simulink model "hcu_main_ADASwEPS"  (Simulink 8.2)
settings: Solver=FixedStepDiscrete  StartTime=0.0  StopTime=inf  FixedStep=0.001  RelTol=1e-3
PostLoadFcn:
  | , if any(exist('dsrtsu_mdlpostloadfcn', 'file') == [2, 3, 6]), try dsrtsu_mdlpostloadfcn('Execute', bdroot); catch fprintf('Error in PostLoadFcn (dsrtsu_mdlpostloadfcn) for model "%s":\n %s\n', bdroot, lasterr); end, end,
values from neighbouring files (symbols this model uses):
  C_TASK_1MS_S = (	C_TICK_TIME_S       )    [hcu_local_hdr.m]    (also in temp_ovrd_values.m = double(	0.001                  ))
  C_TICK_TIME_S = single(	0.005	    	)    [hcu_local_hdr.m]
  ENUM_EPSLFCSTATUS_ACTIVE = uint8(  2  )    [hcu_local_hdr.m]
  ENUM_EPSLFCSTATUS_TRANSITION = uint8(  3  )    [hcu_local_hdr.m]
  ENUM_EPSLKASTATUS_ACTIVE = uint8(  2  )    [hcu_local_hdr.m]
  ENUM_EPSMODEREQ_ANGLE = uint8(  1  )    [hcu_local_hdr.m]
  ENUM_EPSMODEREQ_INTERNAL = uint8(  0  )    [hcu_local_hdr.m]
  ENUM_EPSMODEREQ_TORQUE = uint8(  2  )    [hcu_local_hdr.m]
  ENUM_GEARPOSN_1ST = uint8(  1  )    [hcu_local_hdr.m]
  ENUM_GEARPOSN_2ND = uint8(  2  )    [hcu_local_hdr.m]
  ENUM_GEARPOSN_3RD = uint8(  3  )    [hcu_local_hdr.m]
  ENUM_GEARPOSN_4TH = uint8(  4  )    [hcu_local_hdr.m]
  ENUM_GEARPOSN_5TH = uint8(  5  )    [hcu_local_hdr.m]
  ENUM_GEARPOSN_6TH = uint8(  6  )    [hcu_local_hdr.m]
  ENUM_GEARPOSN_R = uint8(  7  )    [hcu_local_hdr.m]
  FALSE = boolean( 0 )    [hcu_local_hdr.m]
  TRUE = boolean( 1 )    [hcu_local_hdr.m]
undefined symbols (not defined in the file or in its folder): AISP_EPSCurrent_pct, AISP_TqASensorDelta_pct, AISP_TqBSensorDelta_pct, dHAL_IN, hal, INVALID_ABS1_TIMEOUT, INVALID_ABS2_TIMEOUT, INVALID_ABS3_TIMEOUT, INVALID_ABS4_TIMEOUT, INVALID_AC1_TIMEOUT, INVALID_ADASTORQ_REQ, INVALID_BCM1_TIMEOUT, INVALID_BCM2_TIMEOUT, INVALID_BOOSTER_VAC, INVALID_CSW1_TIMEOUT, INVALID_CUR_VEHDECE, INVALID_CURBRAKEDECE_REQ, INVALID_CURSTEERANG_REQ, INVALID_CURSTEERTQ_REQ, INVALID_ECM1_TIMEOUT, INVALID_ECM2_TIMEOUT, INVALID_ECM3_TIMEOUT, INVALID_ECM9_TIMEOUT, INVALID_ENG_TORQUE_FRICTIONAL, INVALID_ENG_TORQUE_INDICATED, INVALID_ENG_TORQUE_INDICATEDCOR, INVALID_ENG_TQ_MAX, INVALID_ENG_TQ_MIN, INVALID_EPAS2_TIMEOUT, INVALID_EPAS3_TIMEOUT, INVALID_EPB1_TIMEOUT, INVALID_EPS_BATTVOLT, INVALID_ESC_BATTVOLT, INVALID_GRADE, INVALID_HCU3_TIMEOUT, INVALID_HCU4_TIMEOUT, INVALID_HMI1_TIMEOUT, INVALID_HMI2_TIMEOUT, INVALID_LAT_ACC, INVALID_LONG_ACC, INVALID_MC_PRESSURE, INVALID_METER1_TIMEOUT, INVALID_METER3_TIMEOUT, INVALID_METER_VEHSPD, INVALID_ODO_METER, INVALID_OUTSIDE_TEMP, INVALID_PARKBRAKEBIND_STAT, INVALID_PEDALTQ_REQ, INVALID_SAS1_TIMEOUT, INVALID_SAS_ANGLE, INVALID_SHIFTER_POSN, INVALID_TCM1_TIMEOUT, INVALID_TCM2_TIMEOUT, INVALID_VCU1_TIMEOUT, INVALID_VCU2_TIMEOUT, INVALID_VEH_CRASH, INVALID_VEH_SPD, INVALID_WHEEL_SPD, INVALID_YAW_RATE, KHAL_MssgIdObj1_num ... (+8)
libraries: simulink x147, hcu_lib x38, rti1401lib_dio_type3 x4, rtimmsu_dsrtlib x3, app x1, rtiethernetudplib x1, rti1401lib_adc_type4 x1, rti1401lib_dac_type3 x1, inp x1, lidr x1, outp x1
(part 5 of 15)

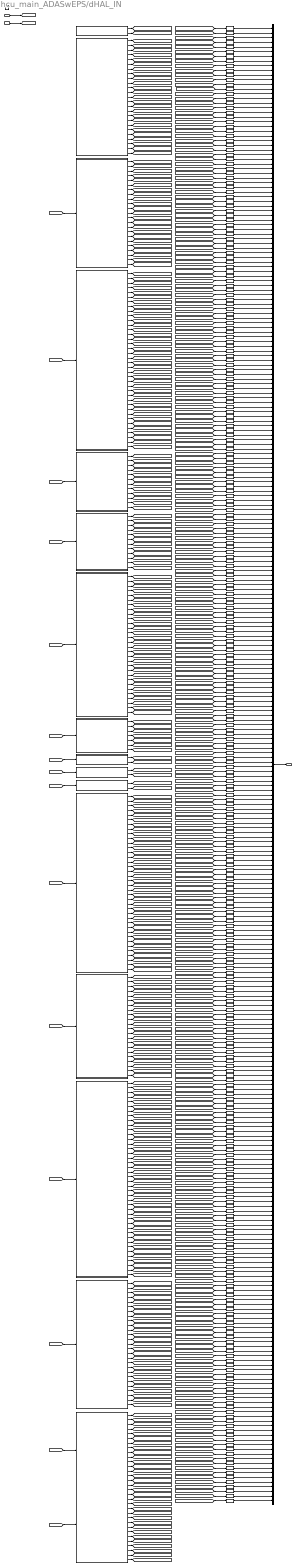
== system hcu_main_ADASwEPS/dHAL_IN ==
  CAN1_Rx : Inport
  CAN2_Rx : Inport  Port=2
  trig_dhal_in : TriggerPort  TriggerType=function-call
  ABS1RollCntCvt : DataTypeConversion  OutDataTypeStr=uint8  SaturateOnIntegerOverflow=on  RndMeth=Zero
  ABS2ChkSumValidCvt : DataTypeConversion  OutDataTypeStr=boolean  SaturateOnIntegerOverflow=on  RndMeth=Zero
  ABS2RollCntCvt : DataTypeConversion  OutDataTypeStr=uint8  SaturateOnIntegerOverflow=on  RndMeth=Zero
  ABSActiveCvt : DataTypeConversion  OutDataTypeStr=boolean  SaturateOnIntegerOverflow=on  RndMeth=Zero
  ABSFaultCvt : DataTypeConversion  OutDataTypeStr=boolean  SaturateOnIntegerOverflow=on  RndMeth=Zero
  ACCCancelHCvt : DataTypeConversion  OutDataTypeStr=boolean  SaturateOnIntegerOverflow=on  RndMeth=Zero
  ACCOnHCvt : DataTypeConversion  OutDataTypeStr=boolean  SaturateOnIntegerOverflow=on  RndMeth=Zero
  ACCOnVCUCvt : DataTypeConversion  OutDataTypeStr=boolean  SaturateOnIntegerOverflow=on  RndMeth=Zero
  ACCResSpdIncHCvt : DataTypeConversion  OutDataTypeStr=boolean  SaturateOnIntegerOverflow=on  RndMeth=Zero
  ACCResSpdIncVCUCvt : DataTypeConversion  OutDataTypeStr=boolean  SaturateOnIntegerOverflow=on  RndMeth=Zero
  ACCSetSpdDecHCvt : DataTypeConversion  OutDataTypeStr=boolean  SaturateOnIntegerOverflow=on  RndMeth=Zero
  ACCSetSpdDecVCUCvt : DataTypeConversion  OutDataTypeStr=boolean  SaturateOnIntegerOverflow=on  RndMeth=Zero
  ACCSpdDecHCvt : DataTypeConversion  OutDataTypeStr=boolean  SaturateOnIntegerOverflow=on  RndMeth=Zero
  ACCSpdIncHCvt : DataTypeConversion  OutDataTypeStr=boolean  SaturateOnIntegerOverflow=on  RndMeth=Zero
  ACCTimeGapDecHCvt : DataTypeConversion  OutDataTypeStr=boolean  SaturateOnIntegerOverflow=on  RndMeth=Zero
  ACCTimeGapDecVCUCvt : DataTypeConversion  OutDataTypeStr=boolean  SaturateOnIntegerOverflow=on  RndMeth=Zero
  ACCTimeGapIncHCvt : DataTypeConversion  OutDataTypeStr=boolean  SaturateOnIntegerOverflow=on  RndMeth=Zero
  ACCTimeGapIncVCUCvt : DataTypeConversion  OutDataTypeStr=boolean  SaturateOnIntegerOverflow=on  RndMeth=Zero
  ADCFaultCvt : DataTypeConversion  OutDataTypeStr=uint8  SaturateOnIntegerOverflow=on  RndMeth=Zero
  AEBEnableHCvt : DataTypeConversion  OutDataTypeStr=boolean  SaturateOnIntegerOverflow=on  RndMeth=Zero
  AccelPedalPosnCvt : DataTypeConversion  OutDataTypeStr=single  SaturateOnIntegerOverflow=on  RndMeth=Zero
  AccelPedalPosnInvalidCvt : DataTypeConversion  OutDataTypeStr=boolean  SaturateOnIntegerOverflow=on  RndMeth=Zero
  AckCurBrakDecReqApplableCvt : DataTypeConversion  OutDataTypeStr=boolean  SaturateOnIntegerOverflow=on  RndMeth=Zero
  AckCurBrakDecReqCvt : DataTypeConversion  OutDataTypeStr=single  SaturateOnIntegerOverflow=on  RndMeth=Zero
  AckCurBrakDecReqInvalidCvt : DataTypeConversion  OutDataTypeStr=boolean  SaturateOnIntegerOverflow=on  RndMeth=Zero
  AckCurPTTqReqApplableCvt : DataTypeConversion  OutDataTypeStr=boolean  SaturateOnIntegerOverflow=on  RndMeth=Zero
  AckCurPTTqReqCvt : DataTypeConversion  OutDataTypeStr=single  SaturateOnIntegerOverflow=on  RndMeth=Zero
  AckCurPTTqReqInvalidCvt : DataTypeConversion  OutDataTypeStr=boolean  SaturateOnIntegerOverflow=on  RndMeth=Zero
  AckCurStrAngReqApplableCvt : DataTypeConversion  OutDataTypeStr=boolean  SaturateOnIntegerOverflow=on  RndMeth=Zero
  AckCurStrAngReqCvt : DataTypeConversion  OutDataTypeStr=single  SaturateOnIntegerOverflow=on  RndMeth=Zero
  AckCurStrAngReqInvalidCvt : DataTypeConversion  OutDataTypeStr=boolean  SaturateOnIntegerOverflow=on  RndMeth=Zero
  AckCurStrTqReqApplableCvt : DataTypeConversion  OutDataTypeStr=boolean  SaturateOnIntegerOverflow=on  RndMeth=Zero
  AckCurStrTqReqCvt : DataTypeConversion  OutDataTypeStr=single  SaturateOnIntegerOverflow=on  RndMeth=Zero
  AckCurStrTqReqInvalidCvt : DataTypeConversion  OutDataTypeStr=boolean  SaturateOnIntegerOverflow=on  RndMeth=Zero
  AckCurVehDecCvt : DataTypeConversion  OutDataTypeStr=single  SaturateOnIntegerOverflow=on  RndMeth=Zero
  AckCurVehDecInvalidCvt : DataTypeConversion  OutDataTypeStr=boolean  SaturateOnIntegerOverflow=on  RndMeth=Zero
  AnyDoorOpenCvt : DataTypeConversion  OutDataTypeStr=boolean  SaturateOnIntegerOverflow=on  RndMeth=Zero
  AppTimeCvt : DataTypeConversion  OutDataTypeStr=single  SaturateOnIntegerOverflow=on  RndMeth=Zero
  BrakBoosterPresCvt : DataTypeConversion  OutDataTypeStr=single  SaturateOnIntegerOverflow=on  RndMeth=Zero
  BrakBoosterPresInvalidCvt : DataTypeConversion  OutDataTypeStr=boolean  SaturateOnIntegerOverflow=on  RndMeth=Zero
  BrkLampOnCvt : DataTypeConversion  OutDataTypeStr=boolean  SaturateOnIntegerOverflow=on  RndMeth=Zero
  BrkLampSigInvalidCvt : DataTypeConversion  OutDataTypeStr=boolean  SaturateOnIntegerOverflow=on  RndMeth=Zero
  BuzzerSwOnFltOpenCircuitCvt : DataTypeConversion  OutDataTypeStr=uint8  SaturateOnIntegerOverflow=on  RndMeth=Zero
  BuzzerSwOnFltShortHighCvt : DataTypeConversion  OutDataTypeStr=uint8  SaturateOnIntegerOverflow=on  RndMeth=Zero
  BuzzerSwOnFltShortLowCvt : DataTypeConversion  OutDataTypeStr=uint8  SaturateOnIntegerOverflow=on  RndMeth=Zero
  CANMsgValidABS1Cvt : DataTypeConversion  OutDataTypeStr=boolean  SaturateOnIntegerOverflow=on  RndMeth=Zero
  CANMsgValidABS2Cvt : DataTypeConversion  OutDataTypeStr=boolean  SaturateOnIntegerOverflow=on  RndMeth=Zero
  CANMsgValidABS3Cvt : DataTypeConversion  OutDataTypeStr=boolean  SaturateOnIntegerOverflow=on  RndMeth=Zero
  CANMsgValidABS4Cvt : DataTypeConversion  OutDataTypeStr=boolean  SaturateOnIntegerOverflow=on  RndMeth=Zero
  CANMsgValidAC1Cvt : DataTypeConversion  OutDataTypeStr=boolean  SaturateOnIntegerOverflow=on  RndMeth=Zero
  CANMsgValidBCM1Cvt : DataTypeConversion  OutDataTypeStr=boolean  SaturateOnIntegerOverflow=on  RndMeth=Zero
  CANMsgValidBCM2Cvt : DataTypeConversion  OutDataTypeStr=boolean  SaturateOnIntegerOverflow=on  RndMeth=Zero
  CANMsgValidECM1Cvt : DataTypeConversion  OutDataTypeStr=boolean  SaturateOnIntegerOverflow=on  RndMeth=Zero
  CANMsgValidECM2Cvt : DataTypeConversion  OutDataTypeStr=boolean  SaturateOnIntegerOverflow=on  RndMeth=Zero
  CANMsgValidECM3Cvt : DataTypeConversion  OutDataTypeStr=boolean  SaturateOnIntegerOverflow=on  RndMeth=Zero
  CANMsgValidECM9Cvt : DataTypeConversion  OutDataTypeStr=boolean  SaturateOnIntegerOverflow=on  RndMeth=Zero
  CANMsgValidEPAS1Cvt : DataTypeConversion  OutDataTypeStr=boolean  SaturateOnIntegerOverflow=on  RndMeth=Zero
  CANMsgValidEPAS2Cvt : DataTypeConversion  OutDataTypeStr=boolean  SaturateOnIntegerOverflow=on  RndMeth=Zero
  CANMsgValidEPAS3Cvt : DataTypeConversion  OutDataTypeStr=boolean  SaturateOnIntegerOverflow=on  RndMeth=Zero
  CANMsgValidEPB1Cvt : DataTypeConversion  OutDataTypeStr=boolean  SaturateOnIntegerOverflow=on  RndMeth=Zero
  CANMsgValidEPB1Cvt1 : DataTypeConversion  OutDataTypeStr=boolean  SaturateOnIntegerOverflow=on  RndMeth=Zero
  CANMsgValidEPM1Cvt : DataTypeConversion  OutDataTypeStr=boolean  SaturateOnIntegerOverflow=on  RndMeth=Zero
  CANMsgValidEPM2Cvt : DataTypeConversion  OutDataTypeStr=boolean  SaturateOnIntegerOverflow=on  RndMeth=Zero
  CANMsgValidEPM3Cvt : DataTypeConversion  OutDataTypeStr=boolean  SaturateOnIntegerOverflow=on  RndMeth=Zero
  CANMsgValidEPM4Cvt : DataTypeConversion  OutDataTypeStr=boolean  SaturateOnIntegerOverflow=on  RndMeth=Zero
  CANMsgValidEPM4Cvt1 : DataTypeConversion  OutDataTypeStr=boolean  SaturateOnIntegerOverflow=on  RndMeth=Zero
  CANMsgValidHCU3Cvt : DataTypeConversion  OutDataTypeStr=boolean  SaturateOnIntegerOverflow=on  RndMeth=Zero
  CANMsgValidHCU4Cvt : DataTypeConversion  OutDataTypeStr=boolean  SaturateOnIntegerOverflow=on  RndMeth=Zero
  CANMsgValidHMI1Cvt : DataTypeConversion  OutDataTypeStr=boolean  SaturateOnIntegerOverflow=on  RndMeth=Zero
  CANMsgValidHMI2Cvt : DataTypeConversion  OutDataTypeStr=boolean  SaturateOnIntegerOverflow=on  RndMeth=Zero
  CANMsgValidMETER1Cvt : DataTypeConversion  OutDataTypeStr=boolean  SaturateOnIntegerOverflow=on  RndMeth=Zero
  CANMsgValidMETER3Cvt : DataTypeConversion  OutDataTypeStr=boolean  SaturateOnIntegerOverflow=on  RndMeth=Zero
  CANMsgValidSAS1Cvt : DataTypeConversion  OutDataTypeStr=boolean  SaturateOnIntegerOverflow=on  RndMeth=Zero
  CANMsgValidTCM1Cvt : DataTypeConversion  OutDataTypeStr=boolean  SaturateOnIntegerOverflow=on  RndMeth=Zero
  CANMsgValidTCM2Cvt : DataTypeConversion  OutDataTypeStr=boolean  SaturateOnIntegerOverflow=on  RndMeth=Zero
  CANMsgValidVCU1Cvt : DataTypeConversion  OutDataTypeStr=boolean  SaturateOnIntegerOverflow=on  RndMeth=Zero
  CANMsgValidVCU2Cvt : DataTypeConversion  OutDataTypeStr=boolean  SaturateOnIntegerOverflow=on  RndMeth=Zero
  CSCEnableHCvt : DataTypeConversion  OutDataTypeStr=boolean  SaturateOnIntegerOverflow=on  RndMeth=Zero
  CurDriverTqReqCvt : DataTypeConversion  OutDataTypeStr=single  SaturateOnIntegerOverflow=on  RndMeth=Zero
  CurDriverTqReqInvalidCvt : DataTypeConversion  OutDataTypeStr=boolean  SaturateOnIntegerOverflow=on  RndMeth=Zero
  CurDriverTqReqInvalidCvt1 : DataTypeConversion  OutDataTypeStr=uint8  SaturateOnIntegerOverflow=on  RndMeth=Zero
  DeceContManagCvt : DataTypeConversion  OutDataTypeStr=boolean  SaturateOnIntegerOverflow=on  RndMeth=Zero
  DefMaxACCSetSpeedCvt : DataTypeConversion  OutDataTypeStr=single  SaturateOnIntegerOverflow=on  RndMeth=Zero
  DriverBrakPedalOnCvt : DataTypeConversion  OutDataTypeStr=boolean  SaturateOnIntegerOverflow=on  RndMeth=Zero
  DriverBrakPedalOnCvt1 : DataTypeConversion  OutDataTypeStr=boolean  SaturateOnIntegerOverflow=on  RndMeth=Zero
  DriverDoorOpenCvt : DataTypeConversion  OutDataTypeStr=boolean  SaturateOnIntegerOverflow=on  RndMeth=Zero
  DriverModeCvt : DataTypeConversion  OutDataTypeStr=uint8  SaturateOnIntegerOverflow=on  RndMeth=Zero
  EBDFaultCvt : DataTypeConversion  OutDataTypeStr=boolean  SaturateOnIntegerOverflow=on  RndMeth=Zero
  ECM9RollCntCvt : DataTypeConversion  OutDataTypeStr=uint8  SaturateOnIntegerOverflow=on  RndMeth=Zero
  ECMExtnTqAvailableCvt : DataTypeConversion  OutDataTypeStr=boolean  SaturateOnIntegerOverflow=on  RndMeth=Zero
  ECMPermMaxTqIndCvt : DataTypeConversion  OutDataTypeStr=boolean  SaturateOnIntegerOverflow=on  RndMeth=Zero
  ECMTqSourceCvt : DataTypeConversion  OutDataTypeStr=uint8  SaturateOnIntegerOverflow=on  RndMeth=Zero
  EEPROMFaultCvt : DataTypeConversion  OutDataTypeStr=uint8  SaturateOnIntegerOverflow=on  RndMeth=Zero
  EMSHybridOpStateCvt : DataTypeConversion  OutDataTypeStr=uint8  SaturateOnIntegerOverflow=on  RndMeth=Zero
  EMSOpStateCvt : DataTypeConversion  OutDataTypeStr=uint8  SaturateOnIntegerOverflow=on  RndMeth=Zero
  EPAS2ChkSumValidCvt : DataTypeConversion  OutDataTypeStr=boolean  SaturateOnIntegerOverflow=on  RndMeth=Zero
  EPAS2RollCntCvt : DataTypeConversion  OutDataTypeStr=uint8  SaturateOnIntegerOverflow=on  RndMeth=Zero
  EPAS3ChkSumValidCvt : DataTypeConversion  OutDataTypeStr=boolean  SaturateOnIntegerOverflow=on  RndMeth=Zero
  EPAS3RollCntCvt{,2..4} (4 alike) : DataTypeConversion  OutDataTypeStr=uint8  SaturateOnIntegerOverflow=on  RndMeth=Zero
  EPASMILReqCvt : DataTypeConversion  OutDataTypeStr=boolean  SaturateOnIntegerOverflow=on  RndMeth=Zero
  EPSBattVoltCvt : DataTypeConversion  OutDataTypeStr=single  SaturateOnIntegerOverflow=on  RndMeth=Zero
  EPSBattVoltInvalidCvt : DataTypeConversion  OutDataTypeStr=boolean  SaturateOnIntegerOverflow=on  RndMeth=Zero
  EPSElectPWRCvt : DataTypeConversion  OutDataTypeStr=single  SaturateOnIntegerOverflow=on  RndMeth=Zero
  EPSFailedCvt : DataTypeConversion  OutDataTypeStr=boolean  SaturateOnIntegerOverflow=on  RndMeth=Zero
  ESCActiveCvt : DataTypeConversion  OutDataTypeStr=boolean  SaturateOnIntegerOverflow=on  RndMeth=Zero
  ESCBattVoltCvt : DataTypeConversion  OutDataTypeStr=single  SaturateOnIntegerOverflow=on  RndMeth=Zero
  ESCBattVoltInvalidCvt : DataTypeConversion  OutDataTypeStr=boolean  SaturateOnIntegerOverflow=on  RndMeth=Zero
  ESCBrakeStatusCvt : DataTypeConversion  OutDataTypeStr=uint8  SaturateOnIntegerOverflow=on  RndMeth=Zero
  ESCExtnBrkAvailableCvt : DataTypeConversion  OutDataTypeStr=boolean  SaturateOnIntegerOverflow=on  RndMeth=Zero
  ESCFaultCvt : DataTypeConversion  OutDataTypeStr=boolean  SaturateOnIntegerOverflow=on  RndMeth=Zero
  EffAccelPedalPosnCvt : DataTypeConversion  OutDataTypeStr=single  SaturateOnIntegerOverflow=on  RndMeth=Zero
  EffAccelPedalPosnInvalidCvt : DataTypeConversion  OutDataTypeStr=boolean  SaturateOnIntegerOverflow=on  RndMeth=Zero
  EngHoodOpenCvt : DataTypeConversion  OutDataTypeStr=boolean  SaturateOnIntegerOverflow=on  RndMeth=Zero
  EngRunningCvt : DataTypeConversion  OutDataTypeStr=boolean  SaturateOnIntegerOverflow=on  RndMeth=Zero
  EngRunningCvt1 : DataTypeConversion  OutDataTypeStr=boolean  SaturateOnIntegerOverflow=on  RndMeth=Zero
  EngSpdCvt : DataTypeConversion  OutDataTypeStr=single  SaturateOnIntegerOverflow=on  RndMeth=Zero
  EngSpdInvalidCvt : DataTypeConversion  OutDataTypeStr=boolean  SaturateOnIntegerOverflow=on  RndMeth=Zero
  EngTqFrictionCvt : DataTypeConversion  OutDataTypeStr=single  SaturateOnIntegerOverflow=on  RndMeth=Zero
  EngTqFrictionInvalidCvt : DataTypeConversion  OutDataTypeStr=boolean  SaturateOnIntegerOverflow=on  RndMeth=Zero
  EngTqIndicatedCORCvt : DataTypeConversion  OutDataTypeStr=single  SaturateOnIntegerOverflow=on  RndMeth=Zero
  EngTqIndicatedCORInvalidCvt : DataTypeConversion  OutDataTypeStr=boolean  SaturateOnIntegerOverflow=on  RndMeth=Zero
  EngTqIndicatedCvt : DataTypeConversion  OutDataTypeStr=single  SaturateOnIntegerOverflow=on  RndMeth=Zero
  EngTqIndicatedInvalidCvt : DataTypeConversion  OutDataTypeStr=boolean  SaturateOnIntegerOverflow=on  RndMeth=Zero
  EngTqMaxCvt : DataTypeConversion  OutDataTypeStr=single  SaturateOnIntegerOverflow=on  RndMeth=Zero
  EngTqMaxInvalidCvt : DataTypeConversion  OutDataTypeStr=boolean  SaturateOnIntegerOverflow=on  RndMeth=Zero
  EngTqMinCvt : DataTypeConversion  OutDataTypeStr=single  SaturateOnIntegerOverflow=on  RndMeth=Zero
  EngTqMinInvalidCvt : DataTypeConversion  OutDataTypeStr=boolean  SaturateOnIntegerOverflow=on  RndMeth=Zero
  EngTqUnCORFaultCvt : DataTypeConversion  OutDataTypeStr=boolean  SaturateOnIntegerOverflow=on  RndMeth=Zero
  FCWEnableHCvt : DataTypeConversion  OutDataTypeStr=boolean  SaturateOnIntegerOverflow=on  RndMeth=Zero
  FCWWarningModeHCvt : DataTypeConversion  OutDataTypeStr=uint8  SaturateOnIntegerOverflow=on  RndMeth=Zero
  HAL_IN_CANVALID : Subsystem
  HAL_IN_CSW : Subsystem
  HAL_IN_EPB : Subsystem
  HAL_IN_EPM : Subsystem
  HAL_IN_HMI : Subsystem
  HAL_IN_RadObjDecoder : Subsystem
  HAL_IN_VCU : Subsystem
  HCU3RollCntCvt : DataTypeConversion  OutDataTypeStr=uint8  SaturateOnIntegerOverflow=on  RndMeth=Zero
  HSAActiveCvt : DataTypeConversion  OutDataTypeStr=boolean  SaturateOnIntegerOverflow=on  RndMeth=Zero
  HSAFaultCvt : DataTypeConversion  OutDataTypeStr=boolean  SaturateOnIntegerOverflow=on  RndMeth=Zero
  HWAccelPedalPosnCvt : DataTypeConversion  OutDataTypeStr=single  SaturateOnIntegerOverflow=on  RndMeth=Zero
  HWAccelPedalPosnInvalidCvt : DataTypeConversion  OutDataTypeStr=boolean  SaturateOnIntegerOverflow=on  RndMeth=Zero
  HazardLightSwCvt : DataTypeConversion  OutDataTypeStr=boolean  SaturateOnIntegerOverflow=on  RndMeth=Zero
  IGSAOnHCvt : DataTypeConversion  OutDataTypeStr=boolean  SaturateOnIntegerOverflow=on  RndMeth=Zero
  IGSAResSpdIncHCvt : DataTypeConversion  OutDataTypeStr=boolean  SaturateOnIntegerOverflow=on  RndMeth=Zero
  IGSASetSpdDecHCvt : DataTypeConversion  OutDataTypeStr=boolean  SaturateOnIntegerOverflow=on  RndMeth=Zero
  IGSASwitchModeHCvt : DataTypeConversion  OutDataTypeStr=boolean  SaturateOnIntegerOverflow=on  RndMeth=Zero
  IgnitionVoltCvt : DataTypeConversion  OutDataTypeStr=single  SaturateOnIntegerOverflow=on  RndMeth=Zero
  KeySwitchStatusCvt : DataTypeConversion  OutDataTypeStr=uint8  SaturateOnIntegerOverflow=on  RndMeth=Zero
  LCSEnableHCvt : DataTypeConversion  OutDataTypeStr=boolean  SaturateOnIntegerOverflow=on  RndMeth=Zero
  LFCOnVCUCvt : DataTypeConversion  OutDataTypeStr=boolean  SaturateOnIntegerOverflow=on  RndMeth=Zero
  LFCPilotCancelHCvt : DataTypeConversion  OutDataTypeStr=boolean  SaturateOnIntegerOverflow=on  RndMeth=Zero
  LFCPilotOnHCvt : DataTypeConversion  OutDataTypeStr=boolean  SaturateOnIntegerOverflow=on  RndMeth=Zero
  LFWheelSpeedCvt : DataTypeConversion  OutDataTypeStr=single  SaturateOnIntegerOverflow=on  RndMeth=Zero
  LFWheelSpeedInvalidCvt : DataTypeConversion  OutDataTypeStr=boolean  SaturateOnIntegerOverflow=on  RndMeth=Zero
  LKAEnableHCvt : DataTypeConversion  OutDataTypeStr=boolean  SaturateOnIntegerOverflow=on  RndMeth=Zero
  LRDoorOpenCvt : DataTypeConversion  OutDataTypeStr=boolean  SaturateOnIntegerOverflow=on  RndMeth=Zero
  LRWheelSpeedCvt : DataTypeConversion  OutDataTypeStr=single  SaturateOnIntegerOverflow=on  RndMeth=Zero
  LRWheelSpeedInvalidCvt : DataTypeConversion  OutDataTypeStr=boolean  SaturateOnIntegerOverflow=on  RndMeth=Zero
  LampBlueOnFltOpenCircuitCvt : DataTypeConversion  OutDataTypeStr=uint8  SaturateOnIntegerOverflow=on  RndMeth=Zero
  LampBlueOnFltShortHighCvt : DataTypeConversion  OutDataTypeStr=uint8  SaturateOnIntegerOverflow=on  RndMeth=Zero
  LampBlueOnFltShortLowCvt : DataTypeConversion  OutDataTypeStr=uint8  SaturateOnIntegerOverflow=on  RndMeth=Zero
  LampGreenOnFltOpenCircuitCvt : DataTypeConversion  OutDataTypeStr=uint8  SaturateOnIntegerOverflow=on  RndMeth=Zero
  LampGreenOnFltShortHighCvt : DataTypeConversion  OutDataTypeStr=uint8  SaturateOnIntegerOverflow=on  RndMeth=Zero
  LampGreenOnFltShortLowCvt : DataTypeConversion  OutDataTypeStr=uint8  SaturateOnIntegerOverflow=on  RndMeth=Zero
  LampRedOnFltOpenCircuitCvt : DataTypeConversion  OutDataTypeStr=uint8  SaturateOnIntegerOverflow=on  RndMeth=Zero
  LampRedOnFltShortHighCvt : DataTypeConversion  OutDataTypeStr=uint8  SaturateOnIntegerOverflow=on  RndMeth=Zero
  LampRedOnFltShortLowCvt : DataTypeConversion  OutDataTypeStr=uint8  SaturateOnIntegerOverflow=on  RndMeth=Zero
  LampYellowOnFltOpenCircuitCvt : DataTypeConversion  OutDataTypeStr=uint8  SaturateOnIntegerOverflow=on  RndMeth=Zero
  LampYellowOnFltShortHighCvt : DataTypeConversion  OutDataTypeStr=uint8  SaturateOnIntegerOverflow=on  RndMeth=Zero
  LampYellowOnFltShortLowCvt : DataTypeConversion  OutDataTypeStr=uint8  SaturateOnIntegerOverflow=on  RndMeth=Zero
  LaneC0LCvt : DataTypeConversion  OutDataTypeStr=single  SaturateOnIntegerOverflow=on  RndMeth=Zero
  LaneC0RCvt : DataTypeConversion  OutDataTypeStr=single  SaturateOnIntegerOverflow=on  RndMeth=Zero
  LaneC1LCvt : DataTypeConversion  OutDataTypeStr=single  SaturateOnIntegerOverflow=on  RndMeth=Zero
  LaneC1RCvt : DataTypeConversion  OutDataTypeStr=single  SaturateOnIntegerOverflow=on  RndMeth=Zero
  LaneC2LCvt : DataTypeConversion  OutDataTypeStr=single  SaturateOnIntegerOverflow=on  RndMeth=Zero
  LaneC2RCvt : DataTypeConversion  OutDataTypeStr=single  SaturateOnIntegerOverflow=on  RndMeth=Zero
  LaneC3LCvt : DataTypeConversion  OutDataTypeStr=single  SaturateOnIntegerOverflow=on  RndMeth=Zero
  LaneC3RCvt : DataTypeConversion  OutDataTypeStr=single  SaturateOnIntegerOverflow=on  RndMeth=Zero
  LaneCrosLCvt : DataTypeConversion  OutDataTypeStr=boolean  SaturateOnIntegerOverflow=on  RndMeth=Zero
  LaneCrosRCvt : DataTypeConversion  OutDataTypeStr=boolean  SaturateOnIntegerOverflow=on  RndMeth=Zero
  LaneMrkClrLCvt : DataTypeConversion  OutDataTypeStr=uint8  SaturateOnIntegerOverflow=on  RndMeth=Zero
  LaneMrkClrRCvt : DataTypeConversion  OutDataTypeStr=uint8  SaturateOnIntegerOverflow=on  RndMeth=Zero
  LaneMrkWidLCvt : DataTypeConversion  OutDataTypeStr=single  SaturateOnIntegerOverflow=on  RndMeth=Zero
  LaneMrkWidRCvt : DataTypeConversion  OutDataTypeStr=single  SaturateOnIntegerOverflow=on  RndMeth=Zero
  LaneQualityLCvt : DataTypeConversion  OutDataTypeStr=uint8  SaturateOnIntegerOverflow=on  RndMeth=Zero
  LaneQualityRCvt : DataTypeConversion  OutDataTypeStr=uint8  SaturateOnIntegerOverflow=on  RndMeth=Zero
  LaneTypeLCvt : DataTypeConversion  OutDataTypeStr=uint8  SaturateOnIntegerOverflow=on  RndMeth=Zero
  LaneTypeRCvt : DataTypeConversion  OutDataTypeStr=uint8  SaturateOnIntegerOverflow=on  RndMeth=Zero
  LatAccelCvt : DataTypeConversion  OutDataTypeStr=single  SaturateOnIntegerOverflow=on  RndMeth=Zero
  LatAccelInvalidCvt : DataTypeConversion  OutDataTypeStr=boolean  SaturateOnIntegerOverflow=on  RndMeth=Zero
  LatDistToborderLeftCvt : DataTypeConversion  OutDataTypeStr=single  SaturateOnIntegerOverflow=on  RndMeth=Zero
  LatDistToborderRightCvt : DataTypeConversion  OutDataTypeStr=single  SaturateOnIntegerOverflow=on  RndMeth=Zero
  LongAccelCvt : DataTypeConversion  OutDataTypeStr=single  SaturateOnIntegerOverflow=on  RndMeth=Zero
  LongAccelInvalidCvt : DataTypeConversion  OutDataTypeStr=boolean  SaturateOnIntegerOverflow=on  RndMeth=Zero
  LowBrakBoosterPresCvt : DataTypeConversion  OutDataTypeStr=boolean  SaturateOnIntegerOverflow=on  RndMeth=Zero
  LowBrakeFluidCvt : DataTypeConversion  OutDataTypeStr=boolean  SaturateOnIntegerOverflow=on  RndMeth=Zero
  MAPAEnableHCvt : DataTypeConversion  OutDataTypeStr=boolean  SaturateOnIntegerOverflow=on  RndMeth=Zero
  MCPressureCvt : DataTypeConversion  OutDataTypeStr=single  SaturateOnIntegerOverflow=on  RndMeth=Zero
  MCPressureInvalidCvt : DataTypeConversion  OutDataTypeStr=boolean  SaturateOnIntegerOverflow=on  RndMeth=Zero
  MILReqCvt : DataTypeConversion  OutDataTypeStr=boolean  SaturateOnIntegerOverflow=on  RndMeth=Zero
  MSAOnVCUCvt : DataTypeConversion  OutDataTypeStr=boolean  SaturateOnIntegerOverflow=on  RndMeth=Zero
  MeasCounterCvt : DataTypeConversion  OutDataTypeStr=uint8  SaturateOnIntegerOverflow=on  RndMeth=Zero
  MeterVehSpdCvt : DataTypeConversion  OutDataTypeStr=single  SaturateOnIntegerOverflow=on  RndMeth=Zero
  MeterVehSpdInvalidCvt : DataTypeConversion  OutDataTypeStr=boolean  SaturateOnIntegerOverflow=on  RndMeth=Zero
  NowGearPosnCvt : DataTypeConversion  OutDataTypeStr=uint8  SaturateOnIntegerOverflow=on  RndMeth=Zero
  NowGearPosnInvalidCvt : DataTypeConversion  OutDataTypeStr=boolean  SaturateOnIntegerOverflow=on  RndMeth=Zero
  OBUBuzzerOnFltOpenCircuitCvt : DataTypeConversion  OutDataTypeStr=uint8  SaturateOnIntegerOverflow=on  RndMeth=Zero
  OBUBuzzerOnFltShortHighCvt : DataTypeConversion  OutDataTypeStr=uint8  SaturateOnIntegerOverflow=on  RndMeth=Zero
  OBUBuzzerOnFltShortLowCvt : DataTypeConversion  OutDataTypeStr=uint8  SaturateOnIntegerOverflow=on  RndMeth=Zero
  OdoMeterCvt : DataTypeConversion  OutDataTypeStr=uint32  SaturateOnIntegerOverflow=on  RndMeth=Zero
  OdoMeterInvalidCvt : DataTypeConversion  OutDataTypeStr=boolean  SaturateOnIntegerOverflow=on  RndMeth=Zero
  OutsideTempCvt : DataTypeConversion  OutDataTypeStr=single  SaturateOnIntegerOverflow=on  RndMeth=Zero
  OutsideTempInvalidCvt : DataTypeConversion  OutDataTypeStr=boolean  SaturateOnIntegerOverflow=on  RndMeth=Zero
  ParkBrakeBindStaCvt : DataTypeConversion  OutDataTypeStr=uint8  SaturateOnIntegerOverflow=on  RndMeth=Zero
  ParkBrakeBindStaInvalidCvt : DataTypeConversion  OutDataTypeStr=boolean  SaturateOnIntegerOverflow=on  RndMeth=Zero
  ParkBrakeBindStaInvalidCvt1 : DataTypeConversion  OutDataTypeStr=boolean  SaturateOnIntegerOverflow=on  RndMeth=Zero
  ParkBrakeBindStaInvalidCvt2 : DataTypeConversion  OutDataTypeStr=boolean  SaturateOnIntegerOverflow=on  RndMeth=Zero
  ParkBrakeOnCvt : DataTypeConversion  OutDataTypeStr=boolean  SaturateOnIntegerOverflow=on  RndMeth=Zero
  PassengerDoorOpenCvt : DataTypeConversion  OutDataTypeStr=boolean  SaturateOnIntegerOverflow=on  RndMeth=Zero
  RAMFaultCvt : DataTypeConversion  OutDataTypeStr=uint8  SaturateOnIntegerOverflow=on  RndMeth=Zero
  RFWheelSpeedCvt : DataTypeConversion  OutDataTypeStr=single  SaturateOnIntegerOverflow=on  RndMeth=Zero
  RFWheelSpeedInvalidCvt : DataTypeConversion  OutDataTypeStr=boolean  SaturateOnIntegerOverflow=on  RndMeth=Zero
  ROMFaultCvt : DataTypeConversion  OutDataTypeStr=uint8  SaturateOnIntegerOverflow=on  RndMeth=Zero
  RRDoorOpenCvt : DataTypeConversion  OutDataTypeStr=boolean  SaturateOnIntegerOverflow=on  RndMeth=Zero
  RRWheelSpeedCvt : DataTypeConversion  OutDataTypeStr=single  SaturateOnIntegerOverflow=on  RndMeth=Zero
  RRWheelSpeedInvalidCvt : DataTypeConversion  OutDataTypeStr=boolean  SaturateOnIntegerOverflow=on  RndMeth=Zero
  RadNofObjectsCvt : DataTypeConversion  OutDataTypeStr=uint8  SaturateOnIntegerOverflow=on  RndMeth=Zero
  RadObjAccelXVect40Cvt : DataTypeConversion  OutDataTypeStr=single  SaturateOnIntegerOverflow=on  RndMeth=Zero
  RadObjDynPropVect40Cvt : DataTypeConversion  OutDataTypeStr=uint8  SaturateOnIntegerOverflow=on  RndMeth=Zero
  RadObjIDVect40Cvt : DataTypeConversion  OutDataTypeStr=uint8  SaturateOnIntegerOverflow=on  RndMeth=Zero
  RadObjLengthVect40Cvt : DataTypeConversion  OutDataTypeStr=single  SaturateOnIntegerOverflow=on  RndMeth=Zero
  RadObjMeasStatVect40Cvt : DataTypeConversion  OutDataTypeStr=uint8  SaturateOnIntegerOverflow=on  RndMeth=Zero
  RadObjPExistVect40Cvt : DataTypeConversion  OutDataTypeStr=uint8  SaturateOnIntegerOverflow=on  RndMeth=Zero
  RadObjProbVect40Cvt : DataTypeConversion  OutDataTypeStr=uint8  SaturateOnIntegerOverflow=on  RndMeth=Zero
  RadObjRCSVect40Cvt : DataTypeConversion  OutDataTypeStr=uint8  SaturateOnIntegerOverflow=on  RndMeth=Zero
  RadObjRolCountVect40Cvt : DataTypeConversion  OutDataTypeStr=uint8  SaturateOnIntegerOverflow=on  RndMeth=Zero
  RadObjVrelXVect40Cvt : DataTypeConversion  OutDataTypeStr=single  SaturateOnIntegerOverflow=on  RndMeth=Zero
  RadObjVrelYVect40Cvt : DataTypeConversion  OutDataTypeStr=single  SaturateOnIntegerOverflow=on  RndMeth=Zero
  RadObjWidthVect40Cvt : DataTypeConversion  OutDataTypeStr=single  SaturateOnIntegerOverflow=on  RndMeth=Zero
  RadObjXDisplVect40Cvt : DataTypeConversion  OutDataTypeStr=single  SaturateOnIntegerOverflow=on  RndMeth=Zero
  RadObjYDisplVect40Cvt : DataTypeConversion  OutDataTypeStr=single  SaturateOnIntegerOverflow=on  RndMeth=Zero
  RadWarningLevelCvt : DataTypeConversion  OutDataTypeStr=uint8  SaturateOnIntegerOverflow=on  RndMeth=Zero
  RadWarningObjIDCvt : DataTypeConversion  OutDataTypeStr=uint8  SaturateOnIntegerOverflow=on  RndMeth=Zero
  RelSteerAngleCvt : DataTypeConversion  OutDataTypeStr=single  SaturateOnIntegerOverflow=on  RndMeth=Zero
  RelSteerAngleInvalidCvt : DataTypeConversion  OutDataTypeStr=boolean  SaturateOnIntegerOverflow=on  RndMeth=Zero
  SAS1ChkSumValidCvt : DataTypeConversion  OutDataTypeStr=boolean  SaturateOnIntegerOverflow=on  RndMeth=Zero
  SAS1RollCntCvt : DataTypeConversion  OutDataTypeStr=uint8  SaturateOnIntegerOverflow=on  RndMeth=Zero
  SASAngleCvt : DataTypeConversion  OutDataTypeStr=single  SaturateOnIntegerOverflow=on  RndMeth=Zero
  SASAngleInvalidCvt : DataTypeConversion  OutDataTypeStr=boolean  SaturateOnIntegerOverflow=on  RndMeth=Zero
  SASCalibratedCvt : DataTypeConversion  OutDataTypeStr=boolean  SaturateOnIntegerOverflow=on  RndMeth=Zero
  SASSensorValidCvt : DataTypeConversion  OutDataTypeStr=boolean  SaturateOnIntegerOverflow=on  RndMeth=Zero
  SASSpeedCvt : DataTypeConversion  OutDataTypeStr=single  SaturateOnIntegerOverflow=on  RndMeth=Zero
  SASSpeedValidCvt : DataTypeConversion  OutDataTypeStr=boolean  SaturateOnIntegerOverflow=on  RndMeth=Zero
  SeatBeltNOTFastenCvt : DataTypeConversion  OutDataTypeStr=boolean  SaturateOnIntegerOverflow=on  RndMeth=Zero
  SensorDefectiveCvt : DataTypeConversion  OutDataTypeStr=uint8  SaturateOnIntegerOverflow=on  RndMeth=Zero
  SensorExternalDisturbedCvt : DataTypeConversion  OutDataTypeStr=uint8  SaturateOnIntegerOverflow=on  RndMeth=Zero
  SensorMisalignedCvt : DataTypeConversion  OutDataTypeStr=uint8  SaturateOnIntegerOverflow=on  RndMeth=Zero
  SensorOutputReducedCvt : DataTypeConversion  OutDataTypeStr=uint8  SaturateOnIntegerOverflow=on  RndMeth=Zero
  SensorRxInvalidCvt : DataTypeConversion  OutDataTypeStr=uint8  SaturateOnIntegerOverflow=on  RndMeth=Zero
  SensorSupplyVoltageCvt : DataTypeConversion  OutDataTypeStr=single  SaturateOnIntegerOverflow=on  RndMeth=Zero
  SensorSwitchedOffCvt : DataTypeConversion  OutDataTypeStr=uint8  SaturateOnIntegerOverflow=on  RndMeth=Zero
  ShifterPosnCvt : DataTypeConversion  OutDataTypeStr=uint8  SaturateOnIntegerOverflow=on  RndMeth=Zero
  ShifterPosnInvalidCvt : DataTypeConversion  OutDataTypeStr=boolean  SaturateOnIntegerOverflow=on  RndMeth=Zero
  SteerTorqueCvt : DataTypeConversion  OutDataTypeStr=single  SaturateOnIntegerOverflow=on  RndMeth=Zero
  SteerTorqueInvalidCvt : DataTypeConversion  OutDataTypeStr=boolean  SaturateOnIntegerOverflow=on  RndMeth=Zero
  SurfaceGradeCvt : DataTypeConversion  OutDataTypeStr=single  SaturateOnIntegerOverflow=on  RndMeth=Zero
  SurfaceGradeInvalidCvt : DataTypeConversion  OutDataTypeStr=boolean  SaturateOnIntegerOverflow=on  RndMeth=Zero
  TCMFaultStatusCvt : DataTypeConversion  OutDataTypeStr=uint8  SaturateOnIntegerOverflow=on  RndMeth=Zero
  TCMFaultStatusCvt1 : DataTypeConversion  OutDataTypeStr=uint8  SaturateOnIntegerOverflow=on  RndMeth=Zero
  TCSActiveCvt : DataTypeConversion  OutDataTypeStr=boolean  SaturateOnIntegerOverflow=on  RndMeth=Zero
  TCSEnabledCvt : DataTypeConversion  OutDataTypeStr=boolean  SaturateOnIntegerOverflow=on  RndMeth=Zero
  TCSFaultCvt : DataTypeConversion  OutDataTypeStr=boolean  SaturateOnIntegerOverflow=on  RndMeth=Zero
  TLCLCvt : DataTypeConversion  OutDataTypeStr=single  SaturateOnIntegerOverflow=on  RndMeth=Zero
  TLCRCvt : DataTypeConversion  OutDataTypeStr=single  SaturateOnIntegerOverflow=on  RndMeth=Zero
  TLCRCvt1 : DataTypeConversion  OutDataTypeStr=uint8  SaturateOnIntegerOverflow=on  RndMeth=Zero
  TLCRCvt{3..18} (16 alike) : DataTypeConversion  OutDataTypeStr=boolean  SaturateOnIntegerOverflow=on  RndMeth=Zero
  TLCRCvt2 : DataTypeConversion  OutDataTypeStr=uint8  SaturateOnIntegerOverflow=on  RndMeth=Zero
  TMTurbineSpdCvt : DataTypeConversion  OutDataTypeStr=single  SaturateOnIntegerOverflow=on  RndMeth=Zero
  TMTurbineSpdInvalidCvt{,1..3} (4 alike) : DataTypeConversion  OutDataTypeStr=boolean  SaturateOnIntegerOverflow=on  RndMeth=Zero
  TailGateOpenCvt : DataTypeConversion  OutDataTypeStr=boolean  SaturateOnIntegerOverflow=on  RndMeth=Zero
  TurnSignalSwLCvt : DataTypeConversion  OutDataTypeStr=boolean  SaturateOnIntegerOverflow=on  RndMeth=Zero
  TurnSignalSwRCvt : DataTypeConversion  OutDataTypeStr=boolean  SaturateOnIntegerOverflow=on  RndMeth=Zero
  VCU1ChkSumValidCvt : DataTypeConversion  OutDataTypeStr=boolean  SaturateOnIntegerOverflow=on  RndMeth=Zero
  VCU1RollCntCvt : DataTypeConversion  OutDataTypeStr=uint8  SaturateOnIntegerOverflow=on  RndMeth=Zero
  VCU2ChkSumValidCvt : DataTypeConversion  OutDataTypeStr=boolean  SaturateOnIntegerOverflow=on  RndMeth=Zero
  VCU2RollCntCvt : DataTypeConversion  OutDataTypeStr=uint8  SaturateOnIntegerOverflow=on  RndMeth=Zero
  VCU2RollCntCvt1 : DataTypeConversion  OutDataTypeStr=uint8  SaturateOnIntegerOverflow=on  RndMeth=Zero
  VCUSysFaultCvt : DataTypeConversion  OutDataTypeStr=boolean  SaturateOnIntegerOverflow=on  RndMeth=Zero
  VREF1FaultCvt : DataTypeConversion  OutDataTypeStr=uint8  SaturateOnIntegerOverflow=on  RndMeth=Zero
  VREF2FaultCvt : DataTypeConversion  OutDataTypeStr=uint8  SaturateOnIntegerOverflow=on  RndMeth=Zero
  VbatprotVoltCvt : DataTypeConversion  OutDataTypeStr=single  SaturateOnIntegerOverflow=on  RndMeth=Zero
  VehCrashedCvt : DataTypeConversion  OutDataTypeStr=boolean  SaturateOnIntegerOverflow=on  RndMeth=Zero
  VehCrashedInvalidCvt : DataTypeConversion  OutDataTypeStr=boolean  SaturateOnIntegerOverflow=on  RndMeth=Zero
  VehSpdCvt : DataTypeConversion  OutDataTypeStr=single  SaturateOnIntegerOverflow=on  RndMeth=Zero
  VehSpdInvalidCvt : DataTypeConversion  OutDataTypeStr=boolean  SaturateOnIntegerOverflow=on  RndMeth=Zero
  ViewRangeLCvt : DataTypeConversion  OutDataTypeStr=single  SaturateOnIntegerOverflow=on  RndMeth=Zero
  ViewRangeLCvt1 : DataTypeConversion  OutDataTypeStr=single  SaturateOnIntegerOverflow=on  RndMeth=Zero
  ViewRangeRCvt : DataTypeConversion  OutDataTypeStr=single  SaturateOnIntegerOverflow=on  RndMeth=Zero
  ViewRangeRCvt1 : DataTypeConversion  OutDataTypeStr=single  SaturateOnIntegerOverflow=on  RndMeth=Zero
  YawRateCvt : DataTypeConversion  OutDataTypeStr=single  SaturateOnIntegerOverflow=on  RndMeth=Zero
  YawRateInvalidCvt : DataTypeConversion  OutDataTypeStr=boolean  SaturateOnIntegerOverflow=on  RndMeth=Zero
  dHAL_IN_ABS : Subsystem
  dHAL_IN_AC : Subsystem
  dHAL_IN_BCM : Subsystem
  dHAL_IN_ECM : Subsystem
  dHAL_IN_EPAS : Subsystem
  dHAL_IN_HWIO : Subsystem
  dHAL_IN_LLSW : Subsystem
  dHAL_IN_METER : Subsystem
  dHAL_IN_TCM : Subsystem
  halbus : BusCreator  Inputs=316  OutDataTypeStr=Bus: BHAL_outputs
  BHAL_outputs : Outport  OutDataTypeStr=Bus: BHAL_outputs
  wires:
  dHAL_IN_HWIO/2(VHAL_VbatprotVolt_V) -> [VHAL_VbatprotVolt_V]
  dHAL_IN_HWIO/1(VHAL_IgnitionVolt_V) -> [VHAL_IgnitionVolt_V]
  dHAL_IN_LLSW/25(VHAL_LampYellowOnFltShortLow_enum) -> [VHAL_LampYellowOnFltShortLow_enum]
  dHAL_IN_LLSW/24(VHAL_LampYellowOnFltShortHigh_enum) -> [VHAL_LampYellowOnFltShortHigh_enum]
  dHAL_IN_LLSW/23(VHAL_LampYellowOnFltOpenCircuit_enum) -> [VHAL_LampYellowOnFltOpenCircuit_enum]
  dHAL_IN_LLSW/22(VHAL_LampGreenOnFltShortLow_enum) -> [VHAL_LampGreenOnFltShortLow_enum]
  dHAL_IN_LLSW/21(VHAL_LampGreenOnFltShortHigh_enum) -> [VHAL_LampGreenOnFltShortHigh_enum]
  dHAL_IN_LLSW/20(VHAL_LampGreenOnFltOpenCircuit_enum) -> [VHAL_LampGreenOnFltOpenCircuit_enum]
  dHAL_IN_LLSW/19(VHAL_LampBuleOnFltShortLow_enum) -> [VHAL_LampBlueOnFltShortLow_enum]
  dHAL_IN_LLSW/18(VHAL_LampBuleOnFltShortHigh_enum) -> [VHAL_LampBlueOnFltShortHigh_enum]
  dHAL_IN_LLSW/17(VHAL_LampBlueOnFltOpenCircuit_enum) -> [VHAL_LampBlueOnFltOpenCircuit_enum]
  dHAL_IN_LLSW/16(VHAL_LampRedOnFltShortLow_enum) -> [VHAL_LampRedOnFltShortLow_enum]
  dHAL_IN_LLSW/15(VHAL_LampRedOnFltShortHigh_enum) -> [VHAL_LampRedOnFltShortHigh_enum]
  dHAL_IN_LLSW/14(VHAL_LampRedOnFltOpenCircuit_enum) -> [VHAL_LampRedOnFltOpenCircuit_enum]
  dHAL_IN_LLSW/13(VHAL_OBUBuzzerOnFltShortLow_enum) -> [VHAL_OBUBuzzerOnFltShortLow_enum]
  dHAL_IN_LLSW/12(VHAL_OBUBuzzerOnFltShortHigh_enum) -> [VHAL_OBUBuzzerOnFltShortHigh_enum]
  dHAL_IN_LLSW/11(VHAL_OBUBuzzerOnFltOpenCircuit_enum) -> [VHAL_OBUBuzzerOnFltOpenCircuit_enum]
  dHAL_IN_LLSW/10(VHAL_BuzzerSwOnFltShortLow_enum) -> [VHAL_BuzzerSwOnFltShortLow_enum]
  dHAL_IN_LLSW/9(VHAL_BuzzerSwOnFltShortHigh_enum) -> [VHAL_BuzzerSwOnFltShortHigh_enum]
  dHAL_IN_LLSW/8(VHAL_BuzzerSwOnFltOpenCircuit_enum) -> [VHAL_BuzzerSwOnFltOpenCircuit_enum]
  dHAL_IN_LLSW/7(VHAL_VREF2Fault_enum) -> [VHAL_VREF2Fault_enum]
  dHAL_IN_LLSW/6(VHAL_VREF1Fault_enum) -> [VHAL_VREF1Fault_enum]
  dHAL_IN_LLSW/5(VHAL_ROMFault_enum) -> [VHAL_ROMFault_enum]
  dHAL_IN_LLSW/4(VHAL_RAMFault_enum) -> [VHAL_RAMFault_enum]
  dHAL_IN_LLSW/3(VHAL_EEPROMFault_enum) -> [VHAL_EEPROMFault_enum]
  dHAL_IN_LLSW/2(VHAL_ADCFault_enum) -> [VHAL_ADCFault_enum]
  dHAL_IN_LLSW/1(VHAL_AppTime_ms) -> [VHAL_AppTime_ms]
  dHAL_IN_ECM/22(VHAL_OBDWarnCycAchiv_flg) -> [VHAL_OBDWarnCycAchiv_flg]
  dHAL_IN_ECM/21(VHAL_EngHoodOpen_flg) -> [VHAL_EngHoodOpen_flg]
  dHAL_IN_ECM/20(VHAL_ECM9RollCnt_cnt) -> [VHAL_ECM9RollCnt_cnt]
  dHAL_IN_ECM/19(VHAL_EMSOpState_enum) -> [VHAL_EMSOpState_enum]
  dHAL_IN_ECM/18(VHAL_EMSHybridOpState_enum) -> [VHAL_EMSHybridOpState_enum]
  dHAL_IN_ECM/17(VHAL_EngTqMinInvalid_flg) -> [VHAL_EngTqMinInvalid_flg]
  dHAL_IN_ECM/16(VHAL_EngTqMin_Nm) -> [VHAL_EngTqMin_Nm]
  dHAL_IN_ECM/15(VHAL_EngTqMaxInvalid_flg) -> [VHAL_EngTqMaxInvalid_flg]
  dHAL_IN_ECM/14(VHAL_EngTqMax_Nm) -> [VHAL_EngTqMax_Nm]
  dHAL_IN_ECM/13(VHAL_EngTqFrictionInvalid_flg) -> [VHAL_EngTqFrictionInvalid_flg]
  dHAL_IN_ECM/12(VHAL_EngTqFriction_Nm) -> [VHAL_EngTqFriction_Nm]
  dHAL_IN_ECM/11(VHAL_EngTqUnCORFault_flg) -> [VHAL_EngTqUnCORFault_flg]
  dHAL_IN_ECM/10(VHAL_EngTqIndicatedCORInvalid_flg) -> [VHAL_EngTqIndicatedCORInvalid_flg]
  dHAL_IN_ECM/9(VHAL_EngTqIndicatedCOR_Nm) -> [VHAL_EngTqIndicatedCOR_Nm]
  dHAL_IN_ECM/8(VHAL_EngTqIndicatedInvalid_flg) -> [VHAL_EngTqIndicatedInvalid_flg]
  dHAL_IN_ECM/7(VHAL_EngTqIndicated_Nm) -> [VHAL_EngTqIndicated_Nm]
  dHAL_IN_ECM/6(VHAL_EngSpdInvalid_flg) -> [VHAL_EngSpdInvalid_flg]
  dHAL_IN_ECM/5(VHAL_EngSpd_rpm) -> [VHAL_EngSpd_erpm]
  dHAL_IN_ECM/4(VHAL_EffAccelPedalPosnInvalid_flg) -> [VHAL_EffAccelPedalPosnInvalid_flg]
  dHAL_IN_ECM/3(VHAL_EffAccelPedalPosn_pct) -> [VHAL_EffAccelPedalPosn_pct]
  dHAL_IN_ECM/2(VHAL_AccelPedalPosnInvalid_flg) -> [VHAL_AccelPedalPosnInvalid_flg]
  dHAL_IN_ECM/1(VHAL_AccelPedalPosn_pct) -> [VHAL_AccelPedalPosn_pct]
  dHAL_IN_ABS/38(VHAL_RRWheelSpeedInvalid_flg) -> [VHAL_RRWheelSpeedInvalid_flg]
  dHAL_IN_ABS/37(VHAL_RRWheelSpeed_kph) -> [VHAL_RRWheelSpeed_kph]
  dHAL_IN_ABS/36(VHAL_RFWheelSpeedInvalid_flg) -> [VHAL_RFWheelSpeedInvalid_flg]
  dHAL_IN_ABS/35(VHAL_RFWheelSpeed_kph) -> [VHAL_RFWheelSpeed_kph]
  dHAL_IN_ABS/34(VHAL_LRWheelSpeedInvalid_flg) -> [VHAL_LRWheelSpeedInvalid_flg]
  dHAL_IN_ABS/33(VHAL_LRWheelSpeed_kph) -> [VHAL_LRWheelSpeed_kph]
  dHAL_IN_ABS/32(VHAL_LFWheelSpeedInvalid_flg) -> [VHAL_LFWheelSpeedInvalid_flg]
  dHAL_IN_ABS/31(VHAL_LFWheelSpeed_kph) -> [VHAL_LFWheelSpeed_kph]
  dHAL_IN_ABS/30(VHAL_ABS1RollCnt_cnt) -> [VHAL_ABS1RollCnt_cnt]
  dHAL_IN_ABS/29(VHAL_LowBrakBoosterPres_flg) -> [VHAL_LowBrakBoosterPres_flg]
  dHAL_IN_ABS/28(VHAL_BrakBoosterPresInvalid_flg) -> [VHAL_BrakBoosterPresInvalid_flg]
  dHAL_IN_ABS/27(VHAL_BrakBoosterPres_kPa) -> [VHAL_BrakBoosterPres_kPa]
  dHAL_IN_ABS/26(VHAL_SurfaceGradeInvalid_flg) -> [VHAL_SurfaceGradeInvalid_flg]
  dHAL_IN_ABS/25(VHAL_SurfaceGrade_deg) -> [VHAL_SurfaceGrade_deg]
  dHAL_IN_ABS/24(VHAL_YawRateInvalid_flg) -> [VHAL_YawRateInvalid_flg]
  dHAL_IN_ABS/23(VHAL_YawRate_degps) -> [VHAL_YawRate_degps]
  dHAL_IN_ABS/22(VHAL_MCPressureInvalid_flg) -> [VHAL_MCPressureInvalid_flg]
  dHAL_IN_ABS/21(VHAL_MCPressure_bar) -> [VHAL_MCPressure_bar]
  dHAL_IN_ABS/20(VHAL_LongAccelInvalid_flg) -> [VHAL_LongAccelInvalid_flg]
  dHAL_IN_ABS/19(VHAL_LongAccel_G) -> [VHAL_LongAccel_G]
  dHAL_IN_ABS/18(VHAL_LatAccelInvalid_flg) -> [VHAL_LatAccelInvalid_flg]
  dHAL_IN_ABS/17(VHAL_LatAccel_G) -> [VHAL_LatAccel_G]
  dHAL_IN_ABS/16(VHAL_ABS2ChkSumValid_flg) -> [VHAL_ABS2ChkSumValid_flg]
  dHAL_IN_ABS/15(VHAL_ABS2RollCnt_cnt) -> [VHAL_ABS2RollCnt_cnt]
  dHAL_IN_ABS/14(VHAL_VehSpdInvalid_flg) -> [VHAL_VehSpdInvalid_flg]
  dHAL_IN_ABS/13(VHAL_VehSpd_kph) -> [VHAL_VehSpd_kph]
  dHAL_IN_ABS/12(VHAL_TCSFault_flg) -> [VHAL_TCSFault_flg]
  dHAL_IN_ABS/11(VHAL_TCSEnabled_flg) -> [VHAL_TCSEnabled_flg]
  dHAL_IN_ABS/10(VHAL_TCSActive_flg) -> [VHAL_TCSActive_flg]
  dHAL_IN_ABS/9(VHAL_HSAFault_flg) -> [VHAL_HSAFault_flg]
  dHAL_IN_ABS/8(VHAL_HSAActive_flg) -> [VHAL_HSAActive_flg]
  dHAL_IN_ABS/7(VHAL_ESCFault_flg) -> [VHAL_ESCFault_flg]
  dHAL_IN_ABS/6(VHAL_ESCActive_flg) -> [VHAL_ESCActive_flg]
  dHAL_IN_ABS/5(VHAL_EBDFault_flg) -> [VHAL_EBDFault_flg]
  dHAL_IN_ABS/4(VHAL_BrkLampSigInvalid_flg) -> [VHAL_BrkLampSigInvalid_flg]
  dHAL_IN_ABS/3(VHAL_BrkLampOn_flg) -> [VHAL_BrkLampOn_flg]
  dHAL_IN_ABS/2(VHAL_ABSFault_flg) -> [VHAL_ABSFault_flg]
  dHAL_IN_ABS/1(VHAL_ABSActive_flg) -> [VHAL_ABSActive_flg]
  dHAL_IN_BCM/12(VHAL_VehCrashedInvalid_flg) -> [VHAL_VehCrashedInvalid_flg]
  dHAL_IN_BCM/11(VHAL_VehCrashed_flg) -> [VHAL_VehCrashed_flg]
  dHAL_IN_BCM/10(VHAL_HazardLightSw_flg) -> [VHAL_HazardLightSw_flg]
  dHAL_IN_BCM/9(VHAL_AnyDoorOpen_flg) -> [VHAL_AnyDoorOpen_flg]
  dHAL_IN_BCM/8(VHAL_TailGateOpen_flg) -> [VHAL_TailGateOpen_flg]
  dHAL_IN_BCM/7(VHAL_RRDoorOpen_flg) -> [VHAL_RRDoorOpen_flg]
  dHAL_IN_BCM/6(VHAL_LRDoorOpen_flg) -> [VHAL_LRDoorOpen_flg]
  dHAL_IN_BCM/5(VHAL_PassengerDoorOpen_flg) -> [VHAL_PassengerDoorOpen_flg]
  dHAL_IN_BCM/4(VHAL_DriverDoorOpen_flg) -> [VHAL_DriverDoorOpen_flg]
  dHAL_IN_BCM/3(VHAL_TurnSignalSwR_flg) -> [VHAL_TurnSignalSwR_flg]
  dHAL_IN_BCM/2(VHAL_TurnSignalSwL_flg) -> [VHAL_TurnSignalSwL_flg]
  dHAL_IN_BCM/1(VHAL_KeySwitchStatus_enum) -> [VHAL_KeySwitchStatus_enum]
  dHAL_IN_TCM/12(VHAL_DriverMode_enum) -> [VHAL_DriverMode_enum]
  dHAL_IN_TCM/11(VHAL_TCMFaultStatus_enum) -> [VHAL_TCMFaultStatus_enum]
  dHAL_IN_TCM/6(VHAL_TMTurbineSpdInvalid_flg) -> [VHAL_TMTurbineSpdInvalid_flg]
  dHAL_IN_TCM/5(VHAL_TMTurbineSpd_rpm) -> [VHAL_TMTurbineSpd_rpm]
  dHAL_IN_TCM/4(VHAL_NowGearPosnInvalid_flg) -> [VHAL_NowGearPosnInvalid_flg]
  dHAL_IN_TCM/3(VHAL_NowGearPosn_enum) -> [VHAL_NowGearPosn_enum]
  dHAL_IN_TCM/2(VHAL_ShifterPosnInvalid_flg) -> [VHAL_ShifterPosnInvalid_flg]
  dHAL_IN_TCM/1(VHAL_ShifterPosn_enum) -> [VHAL_ShifterPosn_enum]
  dHAL_IN_EPAS/30(VHAL_EPAS3RollCnt_cnt) -> [VHAL_EPAS3RollCnt_cnt]
  dHAL_IN_EPAS/29(VHAL_EPAS3ChkSumValid_flg) -> [VHAL_EPAS3ChkSumValid_flg]
  dHAL_IN_EPAS/25(VHAL_EPSBattVoltInvalid_flg) -> [VHAL_EPSBattVoltInvalid_flg]
  dHAL_IN_EPAS/24(VHAL_EPSBattVolt_V) -> [VHAL_EPSBattVolt_V]
  dHAL_IN_EPAS/23(VHAL_AckCurStrTqReqApplable_flg) -> [VHAL_AckCurStrTqReqApplable_flg]
  dHAL_IN_EPAS/22(VHAL_AckCurStrTqReqInvalid_flg) -> [VHAL_AckCurStrTqReqInvalid_flg]
  dHAL_IN_EPAS/21(VHAL_AckCurStrTqReq_Nm) -> [VHAL_AckCurStrTqReq_Nm]
  dHAL_IN_EPAS/20(VHAL_AckCurStrAngReqApplable_flg) -> [VHAL_AckCurStrAngReqApplable_flg]
  dHAL_IN_EPAS/19(VHAL_AckCurStrAngReqInvalid_flg) -> [VHAL_AckCurStrAngReqInvalid_flg]
  dHAL_IN_EPAS/18(VHAL_AckCurStrAngReq_deg) -> [VHAL_AckCurStrAngReq_deg]
  dHAL_IN_EPAS/17(VHAL_EPAS2RollCnt_cnt) -> [VHAL_EPAS2RollCnt_cnt]
  dHAL_IN_EPAS/16(VHAL_EPAS2ChkSumValid_flg) -> [VHAL_EPAS2ChkSumValid_flg]
  dHAL_IN_EPAS/15(VHAL_EPSFailed_flg) -> [VHAL_EPSFailed_flg]
  dHAL_IN_EPAS/14(VHAL_EPSElectPWR_A) -> [VHAL_EPSElectPWR_A]
  dHAL_IN_EPAS/13(VHAL_SteerTorqueInvalid_flg) -> [VHAL_SteerTorqueInvalid_flg]
  dHAL_IN_EPAS/12(VHAL_SteerTorque_Nm) -> [VHAL_SteerTorque_Nm]
  dHAL_IN_EPAS/11(VHAL_RelSteerAngleInvalid_flg) -> [VHAL_RelSteerAngleInvalid_flg]
  dHAL_IN_EPAS/10(VHAL_RelSteerAngle_deg) -> [VHAL_RelSteerAngle_deg]
  dHAL_IN_EPAS/9(VHAL_EPASMILReq_flg) -> [VHAL_EPASMILReq_flg]
  dHAL_IN_EPAS/8(VHAL_SASSpeedValid_flg) -> [VHAL_SASSpeedValid_flg]
  dHAL_IN_EPAS/7(VHAL_SASSpeed_degps) -> [VHAL_SASSpeed_degps]
  dHAL_IN_EPAS/6(VHAL_SAS1RollCnt_cnt) -> [VHAL_SAS1RollCnt_cnt]
  dHAL_IN_EPAS/5(VHAL_SAS1ChkSumValid_flg) -> [VHAL_SAS1ChkSumValid_flg]
  dHAL_IN_EPAS/4(VHAL_SASSensorValid_flg) -> [VHAL_SASSensorValid_flg]
  dHAL_IN_EPAS/3(VHAL_SASCalibrated_flg) -> [VHAL_SASCalibrated_flg]
  dHAL_IN_EPAS/2(VHAL_SASAngleInvalid_flg) -> [VHAL_SASAngleInvalid_flg]
  dHAL_IN_EPAS/1(VHAL_SASAngle_deg) -> [VHAL_SASAngle_deg]
  dHAL_IN_METER/7(VHAL_MeterVehSpdInvalid_flg) -> [VHAL_MeterVehSpdInvalid_flg]
  dHAL_IN_METER/6(VHAL_MeterVehSpd_kph) -> [VHAL_MeterVehSpd_kph]
  dHAL_IN_METER/5(VHAL_SeatBeltNOTFasten_flg) -> [VHAL_SeatBeltNOTFasten_flg]
  dHAL_IN_METER/4(VHAL_ParkBrakeOn_flg) -> [VHAL_ParkBrakeOn_flg]
  dHAL_IN_METER/3(VHAL_LowBrakeFluid_flg) -> [VHAL_LowBrakeFluid_flg]
  dHAL_IN_METER/2(VHAL_OdoMeterInvalid_flg) -> [VHAL_OdoMeterInvalid_flg]
  dHAL_IN_METER/1(VHAL_OdoMeter_km) -> [VHAL_OdoMeter_km]
  dHAL_IN_AC/2(VHAL_OutsideTempInvalid_flg) -> [VHAL_OutsideTempInvalid_flg]
  dHAL_IN_AC/1(VHAL_OutsideTemp_degC) -> [VHAL_OutsideTemp_degC]
  HAL_IN_EPB/2(VHAL_ParkBrakeBindStaInvalid_flg) -> [VHAL_ParkBrakeBindStaInvalid_flg]
  HAL_IN_EPB/1(VHAL_ParkBrakeBindSta_enum) -> [VHAL_ParkBrakeBindSta_enum]
  HAL_IN_VCU/38(VHAL_MSAOnVCU_flg) -> [VHAL_MSAOnVCU_flg]
  HAL_IN_VCU/37(VHAL_LFCOnVCU_flg) -> [VHAL_LFCOnVCU_flg]
  HAL_IN_VCU/36(VHAL_ACCTimeGapDecVCU_flg) -> [VHAL_ACCTimeGapDecVCU_flg]
  HAL_IN_VCU/35(VHAL_ACCTimeGapIncVCU_flg) -> [VHAL_ACCTimeGapIncVCU_flg]
  HAL_IN_VCU/34(VHAL_ACCSetSpdDecVCU_flg) -> [VHAL_ACCSetSpdDecVCU_flg]
  HAL_IN_VCU/33(VHAL_ACCResSpdIncVCU_flg) -> [VHAL_ACCResSpdIncVCU_flg]
  HAL_IN_VCU/32(VHAL_ACCOnVCU_flg) -> [VHAL_ACCOnVCU_flg]
  HAL_IN_VCU/31(VHAL_HCUMILReq_flg) -> [VHAL_HCUMILReq_flg]
  HAL_IN_VCU/30(VHAL_HCU3RollCnt_cnt) -> [VHAL_HCU3RollCnt_cnt]
  HAL_IN_VCU/29(VHAL_HybridLimpHome_flg) -> [VHAL_HybridLimpHome_flg]
  HAL_IN_VCU/28(VHAL_VCU2RollCnt_cnt) -> [VHAL_VCU2RollCnt_cnt]
  HAL_IN_VCU/27(VHAL_VCU2ChkSumValid_flg) -> [VHAL_VCU2ChkSumValid_flg]
  HAL_IN_VCU/24(VHAL_CurDriverTqReqInvalid_flg) -> [VHAL_CurDriverTqReqInvalid_flg]
  HAL_IN_VCU/23(VHAL_CurDriverTqReq_Nm) -> [VHAL_CurDriverTqReq_Nm]
  HAL_IN_VCU/22(VHAL_HWAccelPedalPosnInvalid_flg) -> [VHAL_HWAccelPedalPosnInvalid_flg]
  HAL_IN_VCU/21(VHAL_HWAccelPedalPosn_pct) -> [VHAL_HWAccelPedalPosn_pct]
  HAL_IN_VCU/20(VHAL_VCU1RollCnt_cnt) -> [VHAL_VCU1RollCnt_cnt]
  HAL_IN_VCU/19(VHAL_VCU1ChkSumValid_flg) -> [VHAL_VCU1ChkSumValid_flg]
  HAL_IN_VCU/18(VHAL_ESCBattVoltInvalid_flg) -> [VHAL_ESCBattVoltInvalid_flg]
  HAL_IN_VCU/17(VHAL_ESCBattVolt_V) -> [VHAL_ESCBattVolt_V]
  HAL_IN_VCU/16(VHAL_VCUSysFault_flg) -> [VHAL_VCUSysFault_flg]
  HAL_IN_VCU/15(VHAL_ESCExtnBrkAvailable_flg) -> [VHAL_ESCExtnBrkAvailable_flg]
  HAL_IN_VCU/14(VHAL_ESCBrakeStatus_enum) -> [VHAL_ESCBrakeStatus_enum]
  HAL_IN_VCU/13(VHAL_ECMTqSource_enum) -> [VHAL_ECMTqSource_enum]
  HAL_IN_VCU/12(VHAL_ECMExtnTqAvailable_flg) -> [VHAL_ECMExtnTqAvailable_flg]
  HAL_IN_VCU/10(VHAL_DriverBrakPedalOn_flg) -> [VHAL_DriverBrakPedalOn_flg]
  HAL_IN_VCU/9(VHAL_DeceContManag_flg) -> [VHAL_DeceContManag_flg]
  HAL_IN_VCU/8(VHAL_AckCurVehDecInvalid_flg) -> [VHAL_AckCurVehDecInvalid_flg]
  HAL_IN_VCU/7(VHAL_AckCurVehDec_mps2) -> [VHAL_AckCurVehDec_mps2]
  HAL_IN_VCU/6(VHAL_AckCurPTTqReqApplable_flg) -> [VHAL_AckCurPTTqReqApplable_flg]
  HAL_IN_VCU/5(VHAL_AckCurPTTqReqInvalid_flg) -> [VHAL_AckCurPTTqReqInvalid_flg]
  HAL_IN_VCU/4(VHAL_AckCurPTTqReq_Nm) -> [VHAL_AckCurPTTqReq_Nm]
  HAL_IN_VCU/3(VHAL_AckCurBrakDecReqApplable_flg) -> [VHAL_AckCurBrakDecReqApplable_flg]
  HAL_IN_VCU/2(VHAL_AckCurBrakDecReqInvalid_flg) -> [VHAL_AckCurBrakDecReqInvalid_flg]
  HAL_IN_VCU/1(VHAL_AckCurBrakDecReq_mps2) -> [VHAL_AckCurBrakDecReq_mps2]
  HAL_IN_HMI/22(VHAL_DefMaxACCSetSpeed_kph) -> [VHAL_DefMaxACCSetSpeed_kph]
  HAL_IN_HMI/21(VHAL_FCWWarningModeH_enum) -> [VHAL_FCWWarningModeH_enum]
  HAL_IN_HMI/20(VHAL_IGSASwitchModeH_flg) -> [VHAL_IGSASwitchModeH_flg]
  HAL_IN_HMI/19(VHAL_IGSASetSpdDecH_flg) -> [VHAL_IGSASetSpdDecH_flg]
  HAL_IN_HMI/18(VHAL_IGSAResSpdIncH_flg) -> [VHAL_IGSAResSpdIncH_flg]
  HAL_IN_HMI/17(VHAL_IGSAOnH_flg) -> [VHAL_IGSAOnH_flg]
  HAL_IN_HMI/16(VHAL_ACCTimeGapDecH_flg) -> [VHAL_ACCTimeGapDecH_flg]
  HAL_IN_HMI/15(VHAL_ACCTimeGapIncH_flg) -> [VHAL_ACCTimeGapIncH_flg]
  HAL_IN_HMI/14(VHAL_ACCSpdDecH_flg) -> [VHAL_ACCSpdDecH_flg]
  HAL_IN_HMI/13(VHAL_ACCSpdIncH_flg) -> [VHAL_ACCSpdIncH_flg]
  HAL_IN_HMI/12(VHAL_ACCSetSpdDecH_flg) -> [VHAL_ACCSetSpdDecH_flg]
  HAL_IN_HMI/11(VHAL_ACCResSpdIncH_flg) -> [VHAL_ACCResSpdIncH_flg]
  HAL_IN_HMI/10(VHAL_ACCCancelH_flg) -> [VHAL_ACCCancelH_flg]
  HAL_IN_HMI/9(VHAL_ACCOnH_flg) -> [VHAL_ACCOnH_flg]
  HAL_IN_HMI/8(VHAL_LFCPilotCancelH_flg) -> [VHAL_LFCPilotCancelH_flg]
  HAL_IN_HMI/7(VHAL_LFCPilotOnH_flg) -> [VHAL_LFCPilotOnH_flg]
  HAL_IN_HMI/6(VHAL_LCSEnableH_flg) -> [VHAL_LCSEnableH_flg]
  HAL_IN_HMI/5(VHAL_MAPAEnableH_flg) -> [VHAL_MAPAEnableH_flg]
  HAL_IN_HMI/4(VHAL_LKAEnableH_flg) -> [VHAL_LKAEnableH_flg]
  HAL_IN_HMI/3(VHAL_CSCEnableH_flg) -> [VHAL_CSCEnableH_flg]
  HAL_IN_HMI/2(VHAL_FCWEnableH_flg) -> [VHAL_FCWEnableH_flg]
  HAL_IN_HMI/1(VHAL_AEBEnableH_flg) -> [VHAL_AEBEnableH_flg]
  HAL_IN_EPM/24(VHAL_TLCR_s) -> [VHAL_TLCR_s]
  HAL_IN_EPM/23(VHAL_TLCL_s) -> [VHAL_TLCL_s]
  HAL_IN_EPM/22(VHAL_LaneMrkClrR_enum) -> [VHAL_LaneMrkClrR_enum]
  HAL_IN_EPM/21(VHAL_LaneMrkClrL_enum) -> [VHAL_LaneMrkClrL_enum]
  HAL_IN_EPM/20(VHAL_LaneCrosR_flg) -> [VHAL_LaneCrosR_flg]
  HAL_IN_EPM/19(VHAL_LaneCrosL_flg) -> [VHAL_LaneCrosL_flg]
  HAL_IN_EPM/17(VHAL_ViewRangeStartR_m) -> [VHAL_ViewRangeStartR_m]
  HAL_IN_EPM/14(VHAL_LaneMrkWidR_m) -> [VHAL_LaneMrkWidR_m]
  HAL_IN_EPM/13(VHAL_LaneMrkWidL_m) -> [VHAL_LaneMrkWidL_m]
  HAL_IN_EPM/12(VHAL_LaneTypeR_enum) -> [VHAL_LaneTypeR_enum]
  HAL_IN_EPM/11(VHAL_LaneTypeL_enum) -> [VHAL_LaneTypeL_enum]
  HAL_IN_EPM/10(VHAL_LaneC3R_rat) -> [VHAL_LaneC3R_rat]
  HAL_IN_EPM/9(VHAL_LaneC2R_rat) -> [VHAL_LaneC2R_rat]
  HAL_IN_EPM/8(VHAL_LaneC1R_rad) -> [VHAL_LaneC1R_rad]
  HAL_IN_EPM/7(VHAL_LaneC0R_m) -> [VHAL_LaneC0R_m]
  HAL_IN_EPM/6(VHAL_LaneC3L_rat) -> [VHAL_LaneC3L_rat]
  HAL_IN_EPM/5(VHAL_LaneC2L_rat) -> [VHAL_LaneC2L_rat]
  HAL_IN_EPM/4(VHAL_LaneC1L_rad) -> [VHAL_LaneC1L_rad]
  HAL_IN_EPM/3(VHAL_LaneC0L_m) -> [VHAL_LaneC0L_m]
  HAL_IN_EPM/2(VHAL_LaneQualityR_enum) -> [VHAL_LaneQualityR_enum]
  HAL_IN_EPM/1(VHAL_LaneQualityL_enum) -> [VHAL_LaneQualityL_enum]
  HAL_IN_RadObjDecoder/27(VHAL_RadWarningObjID_num) -> [VHAL_RadWarningObjID_num]
  HAL_IN_RadObjDecoder/26(VHAL_RadWarningLevel_enum) -> [VHAL_RadWarningLevel_enum]
  HAL_IN_RadObjDecoder/25(VHAL_RadObjProbVect40_num) -> [VHAL_RadObjProbVect40_num]
  HAL_IN_RadObjDecoder/24(VHAL_RadObjVrelYVect40_mps) -> [VHAL_RadObjVrelYVect40_mps]
  HAL_IN_RadObjDecoder/23(VHAL_RadObjRCSVect40_num) -> [VHAL_RadObjRCSVect40_num]
  HAL_IN_RadObjDecoder/22(VHAL_RadObjLengthVect40_m) -> [VHAL_RadObjLengthVect40_m]
  HAL_IN_RadObjDecoder/21(VHAL_RadObjWidthVect40_m) -> [VHAL_RadObjWidthVect40_m]
  HAL_IN_RadObjDecoder/20(VHAL_RadObjMeasStatVect40_enum) -> [VHAL_RadObjMeasStatVect40_enum]
  HAL_IN_RadObjDecoder/19(VHAL_RadObjPExistVect40_enum) -> [VHAL_RadObjPExistVect40_enum]
  HAL_IN_RadObjDecoder/18(VHAL_RadObjDynPropVect40_enum) -> [VHAL_RadObjDynPropVect40_enum]
  HAL_IN_RadObjDecoder/17(VHAL_RadObjYDisplVect40_m) -> [VHAL_RadObjYDisplVect40_m]
  HAL_IN_RadObjDecoder/16(VHAL_RadObjAccelXVect40_mps2) -> [VHAL_RadObjAccelXVect40_mps2]
  HAL_IN_RadObjDecoder/15(VHAL_RadObjVrelXVect40_mps) -> [VHAL_RadObjVrelXVect40_mps]
  HAL_IN_RadObjDecoder/14(VHAL_RadObjXDisplVect40_m) -> [VHAL_RadObjXDisplVect40_m]
  HAL_IN_RadObjDecoder/13(VHAL_RadObjIDVect40_num) -> [VHAL_RadObjIDVect40_num]
  HAL_IN_RadObjDecoder/12(VHAL_RadObjRolCountVect40_num) -> [VHAL_RadObjRolCountVect40_num]
  HAL_IN_RadObjDecoder/11(VHAL_LatDistToborderRight_m) -> [VHAL_LatDistToborderRight_m]
  HAL_IN_RadObjDecoder/10(VHAL_LatDistToborderLeft_m) -> [VHAL_LatDistToborderLeft_m]
  HAL_IN_RadObjDecoder/9(VHAL_SensorOutputReduced_enum) -> [VHAL_SensorOutputReduced_enum]
  HAL_IN_RadObjDecoder/8(VHAL_SensorExternalDisturbed_enum) -> [VHAL_SensorExternalDisturbed_enum]
  HAL_IN_RadObjDecoder/7(VHAL_SensorSwitchedOff_enum) -> [VHAL_SensorSwitchedOff_enum]
  HAL_IN_RadObjDecoder/6(VHAL_SensorMisaligned_enum) -> [VHAL_SensorMisaligned_enum]
  HAL_IN_RadObjDecoder/5(VHAL_SensorDefective_enum) -> [VHAL_SensorDefective_enum]
  HAL_IN_RadObjDecoder/4(VHAL_SensorSupplyVoltage_V) -> [VHAL_SensorSupplyVoltage_V]
  HAL_IN_RadObjDecoder/3(VHAL_SensorRxInvalid_enum) -> [VHAL_SensorRxInvalid_enum]
  HAL_IN_RadObjDecoder/2(VHAL_MeasCounter_num) -> [VHAL_MeasCounter_num]
  HAL_IN_RadObjDecoder/1(VHAL_RadNofObjects_num) -> [VHAL_RadNofObjects_num]
  HAL_IN_CANVALID/31(VHAL_CANMsgValidEPM4_flg) -> [VHAL_CANMsgValidEPM4_flg]
  HAL_IN_CANVALID/30(VHAL_CANMsgValidEPM3_flg) -> [VHAL_CANMsgValidEPM3_flg]
  HAL_IN_CANVALID/29(VHAL_CANMsgValidEPM2_flg) -> [VHAL_CANMsgValidEPM2_flg]
  HAL_IN_CANVALID/28(VHAL_CANMsgValidEPM1_flg) -> [VHAL_CANMsgValidEPM1_flg]
  HAL_IN_CANVALID/27(VHAL_CANMsgValidHMI2_flg) -> [VHAL_CANMsgValidHMI2_flg]
  HAL_IN_CANVALID/26(VHAL_CANMsgValidHMI1_flg) -> [VHAL_CANMsgValidHMI1_flg]
  HAL_IN_CANVALID/25(VHAL_CANMsgValidHCU4_flg) -> [VHAL_CANMsgValidHCU4_flg]
  HAL_IN_CANVALID/24(VHAL_CANMsgValidHCU3_flg) -> [VHAL_CANMsgValidHCU3_flg]
  HAL_IN_CANVALID/23(VHAL_CANMsgValidVCU2_flg) -> [VHAL_CANMsgValidVCU2_flg]
  HAL_IN_CANVALID/22(VHAL_CANMsgValidVCU1_flg) -> [VHAL_CANMsgValidVCU1_flg]
  HAL_IN_CANVALID/20(VHAL_CANMsgValidEPB1_flg) -> [VHAL_CANMsgValidEPB1_flg]
  HAL_IN_CANVALID/19(VHAL_CANMsgValidAC1_flg) -> [VHAL_CANMsgValidAC1_flg]
  HAL_IN_CANVALID/18(VHAL_CANMsgValidMETER3_flg) -> [VHAL_CANMsgValidMETER3_flg]
  HAL_IN_CANVALID/17(VHAL_CANMsgValidMETER1_flg) -> [VHAL_CANMsgValidMETER1_flg]
  HAL_IN_CANVALID/16(VHAL_CANMsgValidBCM2_flg) -> [VHAL_CANMsgValidBCM2_flg]
  HAL_IN_CANVALID/15(VHAL_CANMsgValidBCM1_flg) -> [VHAL_CANMsgValidBCM1_flg]
  HAL_IN_CANVALID/14(VHAL_CANMsgValidEPAS3_flg) -> [VHAL_CANMsgValidEPAS3_flg]
  HAL_IN_CANVALID/13(VHAL_CANMsgValidEPAS2_flg) -> [VHAL_CANMsgValidEPAS2_flg]
  HAL_IN_CANVALID/12(VHAL_CANMsgValidEPAS1_flg) -> [VHAL_CANMsgValidEPAS1_flg]
  HAL_IN_CANVALID/11(VHAL_CANMsgValidSAS1_flg) -> [VHAL_CANMsgValidSAS1_flg]
  HAL_IN_CANVALID/10(VHAL_CANMsgValidTCM2_flg) -> [VHAL_CANMsgValidTCM2_flg]
  HAL_IN_CANVALID/9(VHAL_CANMsgValidTCM1_flg) -> [VHAL_CANMsgValidTCM1_flg]
  HAL_IN_CANVALID/8(VHAL_CANMsgValidECM9_flg) -> [VHAL_CANMsgValidECM9_flg]
  HAL_IN_CANVALID/7(VHAL_CANMsgValidECM3_flg) -> [VHAL_CANMsgValidECM3_flg]
  HAL_IN_CANVALID/6(VHAL_CANMsgValidECM2_flg) -> [VHAL_CANMsgValidECM2_flg]
  HAL_IN_CANVALID/5(VHAL_CANMsgValidECM1_flg) -> [VHAL_CANMsgValidECM1_flg]
  HAL_IN_CANVALID/4(VHAL_CANMsgValidABS4_flg) -> [VHAL_CANMsgValidABS4_flg]
  HAL_IN_CANVALID/3(VHAL_CANMsgValidABS3_flg) -> [VHAL_CANMsgValidABS3_flg]
  HAL_IN_CANVALID/2(VHAL_CANMsgValidABS2_flg) -> [VHAL_CANMsgValidABS2_flg]
  HAL_IN_CANVALID/1(VHAL_CANMsgValidABS1_flg) -> [VHAL_CANMsgValidABS1_flg]
  halbus/1 -> BHAL_outputs/1
  CANMsgValidEPM4Cvt/1 -> halbus/316  "VHAL_CANMsgValidEPM5_flg"
  [VHAL_CANMsgValidEPM5_flg] -> CANMsgValidEPM4Cvt/1
  CANMsgValidEPM3Cvt/1 -> halbus/314  "VHAL_CANMsgValidEPM3_flg"
  [VHAL_CANMsgValidEPM3_flg] -> CANMsgValidEPM3Cvt/1
  CANMsgValidEPM2Cvt/1 -> halbus/313  "VHAL_CANMsgValidEPM2_flg"
  [VHAL_CANMsgValidEPM2_flg] -> CANMsgValidEPM2Cvt/1
  CANMsgValidEPM1Cvt/1 -> halbus/312  "VHAL_CANMsgValidEPM1_flg"
  [VHAL_CANMsgValidEPM1_flg] -> CANMsgValidEPM1Cvt/1
  CANMsgValidHMI2Cvt/1 -> halbus/311  "VHAL_CANMsgValidHMI2_flg"
  [VHAL_CANMsgValidHMI2_flg] -> CANMsgValidHMI2Cvt/1
  CANMsgValidHMI1Cvt/1 -> halbus/310  "VHAL_CANMsgValidHMI1_flg"
  [VHAL_CANMsgValidHMI1_flg] -> CANMsgValidHMI1Cvt/1
  CANMsgValidHCU4Cvt/1 -> halbus/309  "VHAL_CANMsgValidHCU4_flg"
  [VHAL_CANMsgValidHCU4_flg] -> CANMsgValidHCU4Cvt/1
  CANMsgValidHCU3Cvt/1 -> halbus/308  "VHAL_CANMsgValidHCU3_flg"
  [VHAL_CANMsgValidHCU3_flg] -> CANMsgValidHCU3Cvt/1
  CANMsgValidVCU2Cvt/1 -> halbus/307  "VHAL_CANMsgValidVCU2_flg"
  [VHAL_CANMsgValidVCU2_flg] -> CANMsgValidVCU2Cvt/1
  CANMsgValidVCU1Cvt/1 -> halbus/306  "VHAL_CANMsgValidVCU1_flg"
  [VHAL_CANMsgValidVCU1_flg] -> CANMsgValidVCU1Cvt/1
  CANMsgValidEPB1Cvt/1 -> halbus/304  "VHAL_CANMsgValidEPB1_flg"
  [VHAL_CANMsgValidEPB1_flg] -> CANMsgValidEPB1Cvt/1
  CANMsgValidAC1Cvt/1 -> halbus/303  "VHAL_CANMsgValidAC1_flg"
  [VHAL_CANMsgValidAC1_flg] -> CANMsgValidAC1Cvt/1
  CANMsgValidMETER3Cvt/1 -> halbus/302  "VHAL_CANMsgValidMETER3_flg"
  [VHAL_CANMsgValidMETER3_flg] -> CANMsgValidMETER3Cvt/1
  CANMsgValidMETER1Cvt/1 -> halbus/301  "VHAL_CANMsgValidMETER1_flg"
  [VHAL_CANMsgValidMETER1_flg] -> CANMsgValidMETER1Cvt/1
  CANMsgValidBCM2Cvt/1 -> halbus/300  "VHAL_CANMsgValidBCM2_flg"
  [VHAL_CANMsgValidBCM2_flg] -> CANMsgValidBCM2Cvt/1
  CANMsgValidBCM1Cvt/1 -> halbus/299  "VHAL_CANMsgValidBCM1_flg"
  [VHAL_CANMsgValidBCM1_flg] -> CANMsgValidBCM1Cvt/1
  CANMsgValidEPAS3Cvt/1 -> halbus/298  "VHAL_CANMsgValidEPAS3_flg"
  [VHAL_CANMsgValidEPAS3_flg] -> CANMsgValidEPAS3Cvt/1
  CANMsgValidEPAS2Cvt/1 -> halbus/297  "VHAL_CANMsgValidEPAS2_flg"
  [VHAL_CANMsgValidEPAS2_flg] -> CANMsgValidEPAS2Cvt/1
  CANMsgValidEPAS1Cvt/1 -> halbus/296  "VHAL_CANMsgValidEPAS1_flg"
  [VHAL_CANMsgValidEPAS1_flg] -> CANMsgValidEPAS1Cvt/1
  CANMsgValidSAS1Cvt/1 -> halbus/295  "VHAL_CANMsgValidSAS1_flg"
  [VHAL_CANMsgValidSAS1_flg] -> CANMsgValidSAS1Cvt/1
  CANMsgValidTCM2Cvt/1 -> halbus/294  "VHAL_CANMsgValidTCM2_flg"
  [VHAL_CANMsgValidTCM2_flg] -> CANMsgValidTCM2Cvt/1
  CANMsgValidTCM1Cvt/1 -> halbus/293  "VHAL_CANMsgValidTCM1_flg"
  [VHAL_CANMsgValidTCM1_flg] -> CANMsgValidTCM1Cvt/1
  CANMsgValidECM9Cvt/1 -> halbus/292  "VHAL_CANMsgValidECM9_flg"
  [VHAL_CANMsgValidECM9_flg] -> CANMsgValidECM9Cvt/1
  CANMsgValidECM3Cvt/1 -> halbus/291  "VHAL_CANMsgValidECM3_flg"
  [VHAL_CANMsgValidECM3_flg] -> CANMsgValidECM3Cvt/1
  CANMsgValidECM2Cvt/1 -> halbus/290  "VHAL_CANMsgValidECM2_flg"
  [VHAL_CANMsgValidECM2_flg] -> CANMsgValidECM2Cvt/1
  CANMsgValidECM1Cvt/1 -> halbus/289  "VHAL_CANMsgValidECM1_flg"
  [VHAL_CANMsgValidECM1_flg] -> CANMsgValidECM1Cvt/1
  CANMsgValidABS4Cvt/1 -> halbus/288  "VHAL_CANMsgValidABS4_flg"
  [VHAL_CANMsgValidABS4_flg] -> CANMsgValidABS4Cvt/1
  CANMsgValidABS3Cvt/1 -> halbus/287  "VHAL_CANMsgValidABS3_flg"
  [VHAL_CANMsgValidABS3_flg] -> CANMsgValidABS3Cvt/1
  CANMsgValidABS2Cvt/1 -> halbus/286  "VHAL_CANMsgValidABS2_flg"
  [VHAL_CANMsgValidABS2_flg] -> CANMsgValidABS2Cvt/1
  CANMsgValidABS1Cvt/1 -> halbus/285  "VHAL_CANMsgValidABS1_flg"
  [VHAL_CANMsgValidABS1_flg] -> CANMsgValidABS1Cvt/1
  RadWarningObjIDCvt/1 -> halbus/284  "VHAL_RadWarningObjID_num"
  [VHAL_RadWarningObjID_num] -> RadWarningObjIDCvt/1
  RadWarningLevelCvt/1 -> halbus/283  "VHAL_RadWarningLevel_enum"
  [VHAL_RadWarningLevel_enum] -> RadWarningLevelCvt/1
  RadObjProbVect40Cvt/1 -> halbus/282  "VHAL_RadObjProbVect40_num"
  [VHAL_RadObjProbVect40_num] -> RadObjProbVect40Cvt/1
  RadObjVrelYVect40Cvt/1 -> halbus/281  "VHAL_RadObjVrelYVect40_mps"
  [VHAL_RadObjVrelYVect40_mps] -> RadObjVrelYVect40Cvt/1
  RadObjRCSVect40Cvt/1 -> halbus/280  "VHAL_RadObjRCSVect40_num"
  [VHAL_RadObjRCSVect40_num] -> RadObjRCSVect40Cvt/1
  RadObjLengthVect40Cvt/1 -> halbus/279  "VHAL_RadObjLengthVect40_m"
  [VHAL_RadObjLengthVect40_m] -> RadObjLengthVect40Cvt/1
  RadObjWidthVect40Cvt/1 -> halbus/278  "VHAL_RadObjWidthVect40_m"
  [VHAL_RadObjWidthVect40_m] -> RadObjWidthVect40Cvt/1
  RadObjMeasStatVect40Cvt/1 -> halbus/277  "VHAL_RadObjMeasStatVect40_enum"
  [VHAL_RadObjMeasStatVect40_enum] -> RadObjMeasStatVect40Cvt/1
  RadObjPExistVect40Cvt/1 -> halbus/276  "VHAL_RadObjPExistVect40_enum"
  [VHAL_RadObjPExistVect40_enum] -> RadObjPExistVect40Cvt/1
  RadObjDynPropVect40Cvt/1 -> halbus/275  "VHAL_RadObjDynPropVect40_enum"
  [VHAL_RadObjDynPropVect40_enum] -> RadObjDynPropVect40Cvt/1
  RadObjYDisplVect40Cvt/1 -> halbus/274  "VHAL_RadObjYDisplVect40_m"
  [VHAL_RadObjYDisplVect40_m] -> RadObjYDisplVect40Cvt/1
  RadObjAccelXVect40Cvt/1 -> halbus/273  "VHAL_RadObjAccelXVect40_mps2"
  [VHAL_RadObjAccelXVect40_mps2] -> RadObjAccelXVect40Cvt/1
  RadObjVrelXVect40Cvt/1 -> halbus/272  "VHAL_RadObjVrelXVect40_mps"
  [VHAL_RadObjVrelXVect40_mps] -> RadObjVrelXVect40Cvt/1
  RadObjXDisplVect40Cvt/1 -> halbus/271  "VHAL_RadObjXDisplVect40_m"
  [VHAL_RadObjXDisplVect40_m] -> RadObjXDisplVect40Cvt/1
  RadObjIDVect40Cvt/1 -> halbus/270  "VHAL_RadObjIDVect40_num"
  [VHAL_RadObjIDVect40_num] -> RadObjIDVect40Cvt/1
  RadObjRolCountVect40Cvt/1 -> halbus/269  "VHAL_RadObjRolCountVect40_num"
  [VHAL_RadObjRolCountVect40_num] -> RadObjRolCountVect40Cvt/1
  LatDistToborderRightCvt/1 -> halbus/268  "VHAL_LatDistToborderRight_m"
  [VHAL_LatDistToborderRight_m] -> LatDistToborderRightCvt/1
  LatDistToborderLeftCvt/1 -> halbus/267  "VHAL_LatDistToborderLeft_m"
  [VHAL_LatDistToborderLeft_m] -> LatDistToborderLeftCvt/1
  SensorOutputReducedCvt/1 -> halbus/266  "VHAL_SensorOutputReduced_enum"
  [VHAL_SensorOutputReduced_enum] -> SensorOutputReducedCvt/1
  SensorExternalDisturbedCvt/1 -> halbus/265  "VHAL_SensorExternalDisturbed_enum"
  [VHAL_SensorExternalDisturbed_enum] -> SensorExternalDisturbedCvt/1
  SensorSwitchedOffCvt/1 -> halbus/264  "VHAL_SensorSwitchedOff_enum"
  [VHAL_SensorSwitchedOff_enum] -> SensorSwitchedOffCvt/1
  SensorMisalignedCvt/1 -> halbus/263  "VHAL_SensorMisaligned_enum"
  [VHAL_SensorMisaligned_enum] -> SensorMisalignedCvt/1
  SensorDefectiveCvt/1 -> halbus/262  "VHAL_SensorDefective_enum"
  [VHAL_SensorDefective_enum] -> SensorDefectiveCvt/1
  SensorSupplyVoltageCvt/1 -> halbus/261  "VHAL_SensorSupplyVoltage_V"
  [VHAL_SensorSupplyVoltage_V] -> SensorSupplyVoltageCvt/1
  SensorRxInvalidCvt/1 -> halbus/260  "VHAL_SensorRxInvalid_enum"
  [VHAL_SensorRxInvalid_enum] -> SensorRxInvalidCvt/1
  MeasCounterCvt/1 -> halbus/259  "VHAL_MeasCounter_num"
  [VHAL_MeasCounter_num] -> MeasCounterCvt/1
  RadNofObjectsCvt/1 -> halbus/258  "VHAL_RadNofObjects_num"
  [VHAL_RadNofObjects_num] -> RadNofObjectsCvt/1
  TLCRCvt/1 -> halbus/239  "VHAL_TLCR_s"
  [VHAL_TLCR_s] -> TLCRCvt/1
  TLCLCvt/1 -> halbus/238  "VHAL_TLCL_s"
  [VHAL_TLCL_s] -> TLCLCvt/1
  LaneMrkClrRCvt/1 -> halbus/237  "VHAL_LaneMrkClrR_enum"
  [VHAL_LaneMrkClrR_enum] -> LaneMrkClrRCvt/1
  LaneMrkClrLCvt/1 -> halbus/236  "VHAL_LaneMrkClrL_enum"
  [VHAL_LaneMrkClrL_enum] -> LaneMrkClrLCvt/1
  LaneCrosRCvt/1 -> halbus/235  "VHAL_LaneCrosR_flg"
  [VHAL_LaneCrosR_flg] -> LaneCrosRCvt/1
  LaneCrosLCvt/1 -> halbus/234  "VHAL_LaneCrosL_flg"
  [VHAL_LaneCrosL_flg] -> LaneCrosLCvt/1
  ViewRangeRCvt/1 -> halbus/232  "VHAL_ViewRangeStartR_m"
  [VHAL_ViewRangeStartR_m] -> ViewRangeRCvt/1
  ViewRangeLCvt/1 -> halbus/230  "VHAL_ViewRangeStartL_m"
  [VHAL_ViewRangeStartL_m] -> ViewRangeLCvt/1
  LaneMrkWidRCvt/1 -> halbus/229  "VHAL_LaneMrkWidR_m"
  [VHAL_LaneMrkWidR_m] -> LaneMrkWidRCvt/1
  LaneMrkWidLCvt/1 -> halbus/228  "VHAL_LaneMrkWidL_m"
  [VHAL_LaneMrkWidL_m] -> LaneMrkWidLCvt/1
  LaneTypeRCvt/1 -> halbus/227  "VHAL_LaneTypeR_enum"
  [VHAL_LaneTypeR_enum] -> LaneTypeRCvt/1
  LaneTypeLCvt/1 -> halbus/226  "VHAL_LaneTypeL_enum"
  [VHAL_LaneTypeL_enum] -> LaneTypeLCvt/1
  LaneC3RCvt/1 -> halbus/225  "VHAL_LaneC3R_rat"
  [VHAL_LaneC3R_rat] -> LaneC3RCvt/1
  LaneC2RCvt/1 -> halbus/224  "VHAL_LaneC2R_rat"
  [VHAL_LaneC2R_rat] -> LaneC2RCvt/1
  LaneC1RCvt/1 -> halbus/223  "VHAL_LaneC1R_rad"
  [VHAL_LaneC1R_rad] -> LaneC1RCvt/1
  LaneC0RCvt/1 -> halbus/222  "VHAL_LaneC0R_m"
  [VHAL_LaneC0R_m] -> LaneC0RCvt/1
  LaneC3LCvt/1 -> halbus/221  "VHAL_LaneC3L_rat"
  [VHAL_LaneC3L_rat] -> LaneC3LCvt/1
  LaneC2LCvt/1 -> halbus/220  "VHAL_LaneC2L_rat"
  [VHAL_LaneC2L_rat] -> LaneC2LCvt/1
  LaneC1LCvt/1 -> halbus/219  "VHAL_LaneC1L_rad"
  [VHAL_LaneC1L_rad] -> LaneC1LCvt/1
  LaneC0LCvt/1 -> halbus/218  "VHAL_LaneC0L_m"
  [VHAL_LaneC0L_m] -> LaneC0LCvt/1
  LaneQualityRCvt/1 -> halbus/217  "VHAL_LaneQualityR_enum"
  [VHAL_LaneQualityR_enum] -> LaneQualityRCvt/1
  LaneQualityLCvt/1 -> halbus/216  "VHAL_LaneQualityL_enum"
  [VHAL_LaneQualityL_enum] -> LaneQualityLCvt/1
  DefMaxACCSetSpeedCvt/1 -> halbus/215  "VHAL_DefMaxACCSetSpeed_kph"
  [VHAL_DefMaxACCSetSpeed_kph] -> DefMaxACCSetSpeedCvt/1
  FCWWarningModeHCvt/1 -> halbus/214  "VHAL_FCWWarningModeH_enum"
  [VHAL_FCWWarningModeH_enum] -> FCWWarningModeHCvt/1
  IGSASwitchModeHCvt/1 -> halbus/213  "VHAL_IGSASwitchModeH_flg"
  [VHAL_IGSASwitchModeH_flg] -> IGSASwitchModeHCvt/1
  IGSASetSpdDecHCvt/1 -> halbus/212  "VHAL_IGSASetSpdDecH_flg"
  [VHAL_IGSASetSpdDecH_flg] -> IGSASetSpdDecHCvt/1
  IGSAResSpdIncHCvt/1 -> halbus/211  "VHAL_IGSAResSpdIncH_flg"
  [VHAL_IGSAResSpdIncH_flg] -> IGSAResSpdIncHCvt/1
  IGSAOnHCvt/1 -> halbus/210  "VHAL_IGSAOnH_flg"
  [VHAL_IGSAOnH_flg] -> IGSAOnHCvt/1
  ACCTimeGapDecHCvt/1 -> halbus/209  "VHAL_ACCTimeGapDecH_flg"
  [VHAL_ACCTimeGapDecH_flg] -> ACCTimeGapDecHCvt/1
  ACCTimeGapIncHCvt/1 -> halbus/208  "VHAL_ACCTimeGapIncH_flg"
  [VHAL_ACCTimeGapIncH_flg] -> ACCTimeGapIncHCvt/1
  ACCSpdDecHCvt/1 -> halbus/207  "VHAL_ACCSpdDecH_flg"
  [VHAL_ACCSpdDecH_flg] -> ACCSpdDecHCvt/1
  ACCSpdIncHCvt/1 -> halbus/206  "VHAL_ACCSpdIncH_flg"
  [VHAL_ACCSpdIncH_flg] -> ACCSpdIncHCvt/1
  ACCSetSpdDecHCvt/1 -> halbus/205  "VHAL_ACCSetSpdDecH_flg"
  [VHAL_ACCSetSpdDecH_flg] -> ACCSetSpdDecHCvt/1
  ACCResSpdIncHCvt/1 -> halbus/204  "VHAL_ACCResSpdIncH_flg"
  [VHAL_ACCResSpdIncH_flg] -> ACCResSpdIncHCvt/1
  ACCCancelHCvt/1 -> halbus/203  "VHAL_ACCCancelH_flg"
  [VHAL_ACCCancelH_flg] -> ACCCancelHCvt/1
  ACCOnHCvt/1 -> halbus/202  "VHAL_ACCOnH_flg"
  [VHAL_ACCOnH_flg] -> ACCOnHCvt/1
  LFCPilotCancelHCvt/1 -> halbus/201  "VHAL_LFCPilotCancelH_flg"
  [VHAL_LFCPilotCancelH_flg] -> LFCPilotCancelHCvt/1
  LFCPilotOnHCvt/1 -> halbus/200  "VHAL_LFCPilotOnH_flg"
  [VHAL_LFCPilotOnH_flg] -> LFCPilotOnHCvt/1
  LCSEnableHCvt/1 -> halbus/199  "VHAL_LCSEnableH_flg"
  [VHAL_LCSEnableH_flg] -> LCSEnableHCvt/1
  MAPAEnableHCvt/1 -> halbus/198  "VHAL_MAPAEnableH_flg"
  [VHAL_MAPAEnableH_flg] -> MAPAEnableHCvt/1
  LKAEnableHCvt/1 -> halbus/197  "VHAL_LKAEnableH_flg"
  [VHAL_LKAEnableH_flg] -> LKAEnableHCvt/1
  CSCEnableHCvt/1 -> halbus/196  "VHAL_CSCEnableH_flg"
  [VHAL_CSCEnableH_flg] -> CSCEnableHCvt/1
  FCWEnableHCvt/1 -> halbus/195  "VHAL_FCWEnableH_flg"
  [VHAL_FCWEnableH_flg] -> FCWEnableHCvt/1
  AEBEnableHCvt/1 -> halbus/194  "VHAL_AEBEnableH_flg"
  [VHAL_AEBEnableH_flg] -> AEBEnableHCvt/1
  MSAOnVCUCvt/1 -> halbus/193  "VHAL_MSAOnVCU_flg"
  [VHAL_MSAOnVCU_flg] -> MSAOnVCUCvt/1
  LFCOnVCUCvt/1 -> halbus/192  "VHAL_LFCOnVCU_flg"
  [VHAL_LFCOnVCU_flg] -> LFCOnVCUCvt/1
  ACCTimeGapDecVCUCvt/1 -> halbus/191  "VHAL_ACCTimeGapDecVCU_flg"
  [VHAL_ACCTimeGapDecVCU_flg] -> ACCTimeGapDecVCUCvt/1
  ACCTimeGapIncVCUCvt/1 -> halbus/190  "VHAL_ACCTimeGapIncVCU_flg"
  [VHAL_ACCTimeGapIncVCU_flg] -> ACCTimeGapIncVCUCvt/1
  ACCSetSpdDecVCUCvt/1 -> halbus/189  "VHAL_ACCSetSpdDecVCU_flg"
  [VHAL_ACCSetSpdDecVCU_flg] -> ACCSetSpdDecVCUCvt/1
  ACCResSpdIncVCUCvt/1 -> halbus/188  "VHAL_ACCResSpdIncVCU_flg"
  [VHAL_ACCResSpdIncVCU_flg] -> ACCResSpdIncVCUCvt/1
  ACCOnVCUCvt/1 -> halbus/187  "VHAL_ACCOnVCU_flg"
  [VHAL_ACCOnVCU_flg] -> ACCOnVCUCvt/1
  MILReqCvt/1 -> halbus/186  "VHAL_HCUMILReq_flg"
  [VHAL_HCUMILReq_flg] -> MILReqCvt/1
  HCU3RollCntCvt/1 -> halbus/185  "VHAL_HCU3RollCnt_cnt"
  [VHAL_HCU3RollCnt_cnt] -> HCU3RollCntCvt/1
  ECMPermMaxTqIndCvt/1 -> halbus/184  "VHAL_HybridLimpHome_flg"
  [VHAL_HybridLimpHome_flg] -> ECMPermMaxTqIndCvt/1
  VCU2RollCntCvt/1 -> halbus/183  "VHAL_VCU2RollCnt_cnt"
  [VHAL_VCU2RollCnt_cnt] -> VCU2RollCntCvt/1
  VCU2ChkSumValidCvt/1 -> halbus/182  "VHAL_VCU2ChkSumValid_flg"
  [VHAL_VCU2ChkSumValid_flg] -> VCU2ChkSumValidCvt/1
  CurDriverTqReqInvalidCvt/1 -> halbus/179  "VHAL_CurDriverTqReqInvalid_flg"
  [VHAL_CurDriverTqReqInvalid_flg] -> CurDriverTqReqInvalidCvt/1
  CurDriverTqReqCvt/1 -> halbus/178  "VHAL_CurDriverTqReq_Nm"
  [VHAL_CurDriverTqReq_Nm] -> CurDriverTqReqCvt/1
  HWAccelPedalPosnInvalidCvt/1 -> halbus/177  "VHAL_HWAccelPedalPosnInvalid_flg"
  [VHAL_HWAccelPedalPosnInvalid_flg] -> HWAccelPedalPosnInvalidCvt/1
  HWAccelPedalPosnCvt/1 -> halbus/176  "VHAL_HWAccelPedalPosn_pct"
  [VHAL_HWAccelPedalPosn_pct] -> HWAccelPedalPosnCvt/1
  VCU1RollCntCvt/1 -> halbus/175  "VHAL_VCU1RollCnt_cnt"
  [VHAL_VCU1RollCnt_cnt] -> VCU1RollCntCvt/1
  VCU1ChkSumValidCvt/1 -> halbus/174  "VHAL_VCU1ChkSumValid_flg"
  [VHAL_VCU1ChkSumValid_flg] -> VCU1ChkSumValidCvt/1
  ESCBattVoltInvalidCvt/1 -> halbus/173  "VHAL_ESCBattVoltInvalid_flg"
  [VHAL_ESCBattVoltInvalid_flg] -> ESCBattVoltInvalidCvt/1
  ESCBattVoltCvt/1 -> halbus/172  "VHAL_ESCBattVolt_V"
  [VHAL_ESCBattVolt_V] -> ESCBattVoltCvt/1
  VCUSysFaultCvt/1 -> halbus/171  "VHAL_VCUSysFault_flg"
  [VHAL_VCUSysFault_flg] -> VCUSysFaultCvt/1
  ESCExtnBrkAvailableCvt/1 -> halbus/170  "VHAL_ESCExtnBrkAvailable_flg"
  [VHAL_ESCExtnBrkAvailable_flg] -> ESCExtnBrkAvailableCvt/1
  ESCBrakeStatusCvt/1 -> halbus/169  "VHAL_ESCBrakeStatus_enum"
  [VHAL_ESCBrakeStatus_enum] -> ESCBrakeStatusCvt/1
  ECMTqSourceCvt/1 -> halbus/168  "VHAL_ECMTqSource_enum"
  [VHAL_ECMTqSource_enum] -> ECMTqSourceCvt/1
  ECMExtnTqAvailableCvt/1 -> halbus/167  "VHAL_ECMExtnTqAvailable_flg"
  [VHAL_ECMExtnTqAvailable_flg] -> ECMExtnTqAvailableCvt/1
  DriverBrakPedalOnCvt/1 -> halbus/165  "VHAL_DriverBrakPedalOn_flg"
  [VHAL_DriverBrakPedalOn_flg] -> DriverBrakPedalOnCvt/1
  DeceContManagCvt/1 -> halbus/164  "VHAL_DeceContManag_flg"
  [VHAL_DeceContManag_flg] -> DeceContManagCvt/1
  AckCurVehDecInvalidCvt/1 -> halbus/163  "VHAL_AckCurVehDecInvalid_flg"
  [VHAL_AckCurVehDecInvalid_flg] -> AckCurVehDecInvalidCvt/1
  AckCurVehDecCvt/1 -> halbus/162  "VHAL_AckCurVehDec_mps2"
  [VHAL_AckCurVehDec_mps2] -> AckCurVehDecCvt/1
  AckCurPTTqReqApplableCvt/1 -> halbus/161  "VHAL_AckCurPTTqReqApplable_flg"
  [VHAL_AckCurPTTqReqApplable_flg] -> AckCurPTTqReqApplableCvt/1
  AckCurPTTqReqInvalidCvt/1 -> halbus/160  "VHAL_AckCurPTTqReqInvalid_flg"
  [VHAL_AckCurPTTqReqInvalid_flg] -> AckCurPTTqReqInvalidCvt/1
  AckCurPTTqReqCvt/1 -> halbus/159  "VHAL_AckCurPTTqReq_Nm"
  [VHAL_AckCurPTTqReq_Nm] -> AckCurPTTqReqCvt/1
  AckCurBrakDecReqApplableCvt/1 -> halbus/158  "VHAL_AckCurBrakDecReqApplable_flg"
  [VHAL_AckCurBrakDecReqApplable_flg] -> AckCurBrakDecReqApplableCvt/1
  AckCurBrakDecReqInvalidCvt/1 -> halbus/157  "VHAL_AckCurBrakDecReqInvalid_flg"
  [VHAL_AckCurBrakDecReqInvalid_flg] -> AckCurBrakDecReqInvalidCvt/1
  AckCurBrakDecReqCvt/1 -> halbus/156  "VHAL_AckCurBrakDecReq_mps2"
  [VHAL_AckCurBrakDecReq_mps2] -> AckCurBrakDecReqCvt/1
  ParkBrakeBindStaInvalidCvt/1 -> halbus/153  "VHAL_ParkBrakeBindStaInvalid_flg"
  [VHAL_ParkBrakeBindStaInvalid_flg] -> ParkBrakeBindStaInvalidCvt/1
  ParkBrakeBindStaCvt/1 -> halbus/152  "VHAL_ParkBrakeBindSta_enum"
  [VHAL_ParkBrakeBindSta_enum] -> ParkBrakeBindStaCvt/1
  OutsideTempInvalidCvt/1 -> halbus/151  "VHAL_OutsideTempInvalid_flg"
  [VHAL_OutsideTempInvalid_flg] -> OutsideTempInvalidCvt/1
  OutsideTempCvt/1 -> halbus/150  "VHAL_OutsideTemp_degC"
  [VHAL_OutsideTemp_degC] -> OutsideTempCvt/1
  MeterVehSpdInvalidCvt/1 -> halbus/149  "VHAL_MeterVehSpdInvalid_flg"
  [VHAL_MeterVehSpdInvalid_flg] -> MeterVehSpdInvalidCvt/1
  MeterVehSpdCvt/1 -> halbus/148  "VHAL_MeterVehSpd_kph"
  [VHAL_MeterVehSpd_kph] -> MeterVehSpdCvt/1
  SeatBeltNOTFastenCvt/1 -> halbus/147  "VHAL_SeatBeltNOTFasten_flg"
  [VHAL_SeatBeltNOTFasten_flg] -> SeatBeltNOTFastenCvt/1
  ParkBrakeOnCvt/1 -> halbus/146  "VHAL_ParkBrakeOn_flg"
  [VHAL_ParkBrakeOn_flg] -> ParkBrakeOnCvt/1
  LowBrakeFluidCvt/1 -> halbus/145  "VHAL_LowBrakeFluid_flg"
  [VHAL_LowBrakeFluid_flg] -> LowBrakeFluidCvt/1
  OdoMeterInvalidCvt/1 -> halbus/144  "VHAL_OdoMeterInvalid_flg"
  [VHAL_OdoMeterInvalid_flg] -> OdoMeterInvalidCvt/1
  OdoMeterCvt/1 -> halbus/143  "VHAL_OdoMeter_km"
  [VHAL_OdoMeter_km] -> OdoMeterCvt/1
  EPAS3RollCntCvt/1 -> halbus/142  "VHAL_EPAS3RollCnt_cnt"
  [VHAL_EPAS3RollCnt_cnt] -> EPAS3RollCntCvt/1
  EPAS3ChkSumValidCvt/1 -> halbus/141  "VHAL_EPAS3ChkSumValid_flg"
  [VHAL_EPAS3ChkSumValid_flg] -> EPAS3ChkSumValidCvt/1
  EPSBattVoltInvalidCvt/1 -> halbus/137  "VHAL_EPSBattVoltInvalid_flg"
  [VHAL_EPSBattVoltInvalid_flg] -> EPSBattVoltInvalidCvt/1
  EPSBattVoltCvt/1 -> halbus/136  "VHAL_EPSBattVolt_V"
  [VHAL_EPSBattVolt_V] -> EPSBattVoltCvt/1
  AckCurStrTqReqApplableCvt/1 -> halbus/135  "VHAL_AckCurStrTqReqApplable_flg"
  [VHAL_AckCurStrTqReqApplable_flg] -> AckCurStrTqReqApplableCvt/1
  AckCurStrTqReqInvalidCvt/1 -> halbus/134  "VHAL_AckCurStrTqReqInvalid_flg"
  [VHAL_AckCurStrTqReqInvalid_flg] -> AckCurStrTqReqInvalidCvt/1
  AckCurStrTqReqCvt/1 -> halbus/133  "VHAL_AckCurStrTqReq_Nm"
  [VHAL_AckCurStrTqReq_Nm] -> AckCurStrTqReqCvt/1
  AckCurStrAngReqApplableCvt/1 -> halbus/132  "VHAL_AckCurStrAngReqApplable_flg"
  [VHAL_AckCurStrAngReqApplable_flg] -> AckCurStrAngReqApplableCvt/1
  AckCurStrAngReqInvalidCvt/1 -> halbus/131  "VHAL_AckCurStrAngReqInvalid_flg"
  [VHAL_AckCurStrAngReqInvalid_flg] -> AckCurStrAngReqInvalidCvt/1
  AckCurStrAngReqCvt/1 -> halbus/130  "VHAL_AckCurStrAngReq_deg"
  [VHAL_AckCurStrAngReq_deg] -> AckCurStrAngReqCvt/1
  EPAS2RollCntCvt/1 -> halbus/129  "VHAL_EPAS2RollCnt_cnt"
  [VHAL_EPAS2RollCnt_cnt] -> EPAS2RollCntCvt/1
  EPAS2ChkSumValidCvt/1 -> halbus/128  "VHAL_EPAS2ChkSumValid_flg"
  [VHAL_EPAS2ChkSumValid_flg] -> EPAS2ChkSumValidCvt/1
  EPSFailedCvt/1 -> halbus/127  "VHAL_EPSFailed_flg"
  [VHAL_EPSFailed_flg] -> EPSFailedCvt/1
  EPSElectPWRCvt/1 -> halbus/126  "VHAL_EPSElectPWR_A"
  [VHAL_EPSElectPWR_A] -> EPSElectPWRCvt/1
  SteerTorqueInvalidCvt/1 -> halbus/125  "VHAL_SteerTorqueInvalid_flg"
  [VHAL_SteerTorqueInvalid_flg] -> SteerTorqueInvalidCvt/1
  SteerTorqueCvt/1 -> halbus/124  "VHAL_SteerTorque_Nm"
  [VHAL_SteerTorque_Nm] -> SteerTorqueCvt/1
  RelSteerAngleInvalidCvt/1 -> halbus/123  "VHAL_RelSteerAngleInvalid_flg"
  [VHAL_RelSteerAngleInvalid_flg] -> RelSteerAngleInvalidCvt/1
  RelSteerAngleCvt/1 -> halbus/122  "VHAL_RelSteerAngle_deg"
  [VHAL_RelSteerAngle_deg] -> RelSteerAngleCvt/1
  EPASMILReqCvt/1 -> halbus/121  "VHAL_EPASMILReq_flg"
  [VHAL_EPASMILReq_flg] -> EPASMILReqCvt/1
  SASSpeedValidCvt/1 -> halbus/120  "VHAL_SASSpeedValid_flg"
  [VHAL_SASSpeedValid_flg] -> SASSpeedValidCvt/1
  SASSpeedCvt/1 -> halbus/119  "VHAL_SASSpeed_degps"
  [VHAL_SASSpeed_degps] -> SASSpeedCvt/1
  SAS1RollCntCvt/1 -> halbus/118  "VHAL_SAS1RollCnt_cnt"
  [VHAL_SAS1RollCnt_cnt] -> SAS1RollCntCvt/1
  SAS1ChkSumValidCvt/1 -> halbus/117  "VHAL_SAS1ChkSumValid_flg"
  [VHAL_SAS1ChkSumValid_flg] -> SAS1ChkSumValidCvt/1
  SASSensorValidCvt/1 -> halbus/116  "VHAL_SASSensorValid_flg"
  [VHAL_SASSensorValid_flg] -> SASSensorValidCvt/1
  SASCalibratedCvt/1 -> halbus/115  "VHAL_SASCalibrated_flg"
  [VHAL_SASCalibrated_flg] -> SASCalibratedCvt/1
  SASAngleInvalidCvt/1 -> halbus/114  "VHAL_SASAngleInvalid_flg"
  [VHAL_SASAngleInvalid_flg] -> SASAngleInvalidCvt/1
  SASAngleCvt/1 -> halbus/113  "VHAL_SASAngle_deg"
  [VHAL_SASAngle_deg] -> SASAngleCvt/1
  DriverModeCvt/1 -> halbus/112  "VHAL_DriverMode_enum"
  [VHAL_DriverMode_enum] -> DriverModeCvt/1
  TCMFaultStatusCvt/1 -> halbus/111  "VHAL_TCMFaultStatus_enum"
  [VHAL_TCMFaultStatus_enum] -> TCMFaultStatusCvt/1
  TMTurbineSpdInvalidCvt/1 -> halbus/106  "VHAL_TMTurbineSpdInvalid_flg"
  [VHAL_TMTurbineSpdInvalid_flg] -> TMTurbineSpdInvalidCvt/1
  TMTurbineSpdCvt/1 -> halbus/105  "VHAL_TMTurbineSpd_rpm"
  [VHAL_TMTurbineSpd_rpm] -> TMTurbineSpdCvt/1
  NowGearPosnInvalidCvt/1 -> halbus/104  "VHAL_NowGearPosnInvalid_flg"
  [VHAL_NowGearPosnInvalid_flg] -> NowGearPosnInvalidCvt/1
  NowGearPosnCvt/1 -> halbus/103  "VHAL_NowGearPosn_enum"
  [VHAL_NowGearPosn_enum] -> NowGearPosnCvt/1
  ShifterPosnInvalidCvt/1 -> halbus/102  "VHAL_ShifterPosnInvalid_flg"
  [VHAL_ShifterPosnInvalid_flg] -> ShifterPosnInvalidCvt/1
  ShifterPosnCvt/1 -> halbus/101  "VHAL_ShifterPosn_enum"
  [VHAL_ShifterPosn_enum] -> ShifterPosnCvt/1
  VehCrashedInvalidCvt/1 -> halbus/100  "VHAL_VehCrashedInvalid_flg"
  [VHAL_VehCrashedInvalid_flg] -> VehCrashedInvalidCvt/1
  VehCrashedCvt/1 -> halbus/99  "VHAL_VehCrashed_flg"
  [VHAL_VehCrashed_flg] -> VehCrashedCvt/1
  HazardLightSwCvt/1 -> halbus/98  "VHAL_HazardLightSw_flg"
  [VHAL_HazardLightSw_flg] -> HazardLightSwCvt/1
  AnyDoorOpenCvt/1 -> halbus/97  "VHAL_AnyDoorOpen_flg"
  [VHAL_AnyDoorOpen_flg] -> AnyDoorOpenCvt/1
  TailGateOpenCvt/1 -> halbus/96  "VHAL_TailGateOpen_flg"
  [VHAL_TailGateOpen_flg] -> TailGateOpenCvt/1
  RRDoorOpenCvt/1 -> halbus/95  "VHAL_RRDoorOpen_flg"
  [VHAL_RRDoorOpen_flg] -> RRDoorOpenCvt/1
  LRDoorOpenCvt/1 -> halbus/94  "VHAL_LRDoorOpen_flg"
  [VHAL_LRDoorOpen_flg] -> LRDoorOpenCvt/1
  PassengerDoorOpenCvt/1 -> halbus/93  "VHAL_PassengerDoorOpen_flg"
  [VHAL_PassengerDoorOpen_flg] -> PassengerDoorOpenCvt/1
  DriverDoorOpenCvt/1 -> halbus/92  "VHAL_DriverDoorOpen_flg"
  [VHAL_DriverDoorOpen_flg] -> DriverDoorOpenCvt/1
  TurnSignalSwRCvt/1 -> halbus/91  "VHAL_TurnSignalSwR_flg"
  [VHAL_TurnSignalSwR_flg] -> TurnSignalSwRCvt/1
  TurnSignalSwLCvt/1 -> halbus/90  "VHAL_TurnSignalSwL_flg"
  [VHAL_TurnSignalSwL_flg] -> TurnSignalSwLCvt/1
  KeySwitchStatusCvt/1 -> halbus/89  "VHAL_KeySwitchStatus_enum"
  [VHAL_KeySwitchStatus_enum] -> KeySwitchStatusCvt/1
  RRWheelSpeedInvalidCvt/1 -> halbus/88  "VHAL_RRWheelSpeedInvalid_flg"
  [VHAL_RRWheelSpeedInvalid_flg] -> RRWheelSpeedInvalidCvt/1
  RRWheelSpeedCvt/1 -> halbus/87  "VHAL_RRWheelSpeed_kph"
  [VHAL_RRWheelSpeed_kph] -> RRWheelSpeedCvt/1
  RFWheelSpeedInvalidCvt/1 -> halbus/86  "VHAL_RFWheelSpeedInvalid_flg"
  [VHAL_RFWheelSpeedInvalid_flg] -> RFWheelSpeedInvalidCvt/1
  RFWheelSpeedCvt/1 -> halbus/85  "VHAL_RFWheelSpeed_kph"
  [VHAL_RFWheelSpeed_kph] -> RFWheelSpeedCvt/1
  LRWheelSpeedInvalidCvt/1 -> halbus/84  "VHAL_LRWheelSpeedInvalid_flg"
  [VHAL_LRWheelSpeedInvalid_flg] -> LRWheelSpeedInvalidCvt/1
  LRWheelSpeedCvt/1 -> halbus/83  "VHAL_LRWheelSpeed_kph"
  [VHAL_LRWheelSpeed_kph] -> LRWheelSpeedCvt/1
  LFWheelSpeedInvalidCvt/1 -> halbus/82  "VHAL_LFWheelSpeedInvalid_flg"
  [VHAL_LFWheelSpeedInvalid_flg] -> LFWheelSpeedInvalidCvt/1
  LFWheelSpeedCvt/1 -> halbus/81  "VHAL_LFWheelSpeed_kph"
  [VHAL_LFWheelSpeed_kph] -> LFWheelSpeedCvt/1
  ABS1RollCntCvt/1 -> halbus/80  "VHAL_ABS1RollCnt_cnt"
  [VHAL_ABS1RollCnt_cnt] -> ABS1RollCntCvt/1
  LowBrakBoosterPresCvt/1 -> halbus/79  "VHAL_LowBrakBoosterPres_flg"
  [VHAL_LowBrakBoosterPres_flg] -> LowBrakBoosterPresCvt/1
  BrakBoosterPresInvalidCvt/1 -> halbus/78  "VHAL_BrakBoosterPresInvalid_flg"
  [VHAL_BrakBoosterPresInvalid_flg] -> BrakBoosterPresInvalidCvt/1
  BrakBoosterPresCvt/1 -> halbus/77  "VHAL_BrakBoosterPres_kPa"
  [VHAL_BrakBoosterPres_kPa] -> BrakBoosterPresCvt/1
  SurfaceGradeInvalidCvt/1 -> halbus/76  "VHAL_SurfaceGradeInvalid_flg"
  [VHAL_SurfaceGradeInvalid_flg] -> SurfaceGradeInvalidCvt/1
  SurfaceGradeCvt/1 -> halbus/75  "VHAL_SurfaceGrade_deg"
  [VHAL_SurfaceGrade_deg] -> SurfaceGradeCvt/1
  YawRateInvalidCvt/1 -> halbus/74  "VHAL_YawRateInvalid_flg"
  [VHAL_YawRateInvalid_flg] -> YawRateInvalidCvt/1
  YawRateCvt/1 -> halbus/73  "VHAL_YawRate_degps"
  [VHAL_YawRate_degps] -> YawRateCvt/1
  MCPressureInvalidCvt/1 -> halbus/72  "VHAL_MCPressureInvalid_flg"
  [VHAL_MCPressureInvalid_flg] -> MCPressureInvalidCvt/1
  MCPressureCvt/1 -> halbus/71  "VHAL_MCPressure_bar"
  [VHAL_MCPressure_bar] -> MCPressureCvt/1
  LongAccelInvalidCvt/1 -> halbus/70  "VHAL_LongAccelInvalid_flg"
  [VHAL_LongAccelInvalid_flg] -> LongAccelInvalidCvt/1
  LongAccelCvt/1 -> halbus/69  "VHAL_LongAccel_G"
  [VHAL_LongAccel_G] -> LongAccelCvt/1
  LatAccelInvalidCvt/1 -> halbus/68  "VHAL_LatAccelInvalid_flg"
  [VHAL_LatAccelInvalid_flg] -> LatAccelInvalidCvt/1
  LatAccelCvt/1 -> halbus/67  "VHAL_LatAccel_G"
  [VHAL_LatAccel_G] -> LatAccelCvt/1
  ABS2ChkSumValidCvt/1 -> halbus/66  "VHAL_ABS2ChkSumValid_flg"
  [VHAL_ABS2ChkSumValid_flg] -> ABS2ChkSumValidCvt/1
  ABS2RollCntCvt/1 -> halbus/65  "VHAL_ABS2RollCnt_cnt"
  [VHAL_ABS2RollCnt_cnt] -> ABS2RollCntCvt/1
  VehSpdInvalidCvt/1 -> halbus/64  "VHAL_VehSpdInvalid_flg"
  [VHAL_VehSpdInvalid_flg] -> VehSpdInvalidCvt/1
  VehSpdCvt/1 -> halbus/63  "VHAL_VehSpd_kph"
  [VHAL_VehSpd_kph] -> VehSpdCvt/1
  TCSFaultCvt/1 -> halbus/62  "VHAL_TCSFault_flg"
  [VHAL_TCSFault_flg] -> TCSFaultCvt/1
  TCSEnabledCvt/1 -> halbus/61  "VHAL_TCSEnabled_flg"
  [VHAL_TCSEnabled_flg] -> TCSEnabledCvt/1
  TCSActiveCvt/1 -> halbus/60  "VHAL_TCSActive_flg"
  [VHAL_TCSActive_flg] -> TCSActiveCvt/1
  HSAFaultCvt/1 -> halbus/59  "VHAL_HSAFault_flg"
  [VHAL_HSAFault_flg] -> HSAFaultCvt/1
  HSAActiveCvt/1 -> halbus/58  "VHAL_HSAActive_flg"
  [VHAL_HSAActive_flg] -> HSAActiveCvt/1
  ESCFaultCvt/1 -> halbus/57  "VHAL_ESCFault_flg"
  [VHAL_ESCFault_flg] -> ESCFaultCvt/1
  ESCActiveCvt/1 -> halbus/56  "VHAL_ESCActive_flg"
  [VHAL_ESCActive_flg] -> ESCActiveCvt/1
  EBDFaultCvt/1 -> halbus/55  "VHAL_EBDFault_flg"
  [VHAL_EBDFault_flg] -> EBDFaultCvt/1
  BrkLampSigInvalidCvt/1 -> halbus/54  "VHAL_BrkLampSigInvalid_flg"
  [VHAL_BrkLampSigInvalid_flg] -> BrkLampSigInvalidCvt/1
  BrkLampOnCvt/1 -> halbus/53  "VHAL_BrkLampOn_flg"
  [VHAL_BrkLampOn_flg] -> BrkLampOnCvt/1
  ABSFaultCvt/1 -> halbus/52  "VHAL_ABSFault_flg"
  [VHAL_ABSFault_flg] -> ABSFaultCvt/1
  ABSActiveCvt/1 -> halbus/51  "VHAL_ABSActive_flg"
  [VHAL_ABSActive_flg] -> ABSActiveCvt/1
  EngRunningCvt/1 -> halbus/49  "VHAL_OBDWarnCycAchiv_flg"
  [VHAL_OBDWarnCycAchiv_flg] -> EngRunningCvt/1
  EngHoodOpenCvt/1 -> halbus/48  "VHAL_EngHoodOpen_flg"
  [VHAL_EngHoodOpen_flg] -> EngHoodOpenCvt/1
  ECM9RollCntCvt/1 -> halbus/47  "VHAL_ECM9RollCnt_cnt"
  [VHAL_ECM9RollCnt_cnt] -> ECM9RollCntCvt/1
  EMSOpStateCvt/1 -> halbus/46  "VHAL_EMSOpState_enum"
  [VHAL_EMSOpState_enum] -> EMSOpStateCvt/1
  EMSHybridOpStateCvt/1 -> halbus/45  "VHAL_EMSHybridOpState_enum"
  [VHAL_EMSHybridOpState_enum] -> EMSHybridOpStateCvt/1
  EngTqMinInvalidCvt/1 -> halbus/44  "VHAL_EngTqMinInvalid_flg"
  [VHAL_EngTqMinInvalid_flg] -> EngTqMinInvalidCvt/1
  EngTqMinCvt/1 -> halbus/43  "VHAL_EngTqMin_Nm"
  [VHAL_EngTqMin_Nm] -> EngTqMinCvt/1
  EngTqMaxInvalidCvt/1 -> halbus/42  "VHAL_EngTqMaxInvalid_flg"
  [VHAL_EngTqMaxInvalid_flg] -> EngTqMaxInvalidCvt/1
  EngTqMaxCvt/1 -> halbus/41  "VHAL_EngTqMax_Nm"
  [VHAL_EngTqMax_Nm] -> EngTqMaxCvt/1
  EngTqFrictionInvalidCvt/1 -> halbus/40  "VHAL_EngTqFrictionInvalid_flg"
  [VHAL_EngTqFrictionInvalid_flg] -> EngTqFrictionInvalidCvt/1
  EngTqFrictionCvt/1 -> halbus/39  "VHAL_EngTqFriction_Nm"
  [VHAL_EngTqFriction_Nm] -> EngTqFrictionCvt/1
  EngTqUnCORFaultCvt/1 -> halbus/38  "VHAL_EngTqUnCORFault_flg"
  [VHAL_EngTqUnCORFault_flg] -> EngTqUnCORFaultCvt/1
  EngTqIndicatedCORInvalidCvt/1 -> halbus/37  "VHAL_EngTqIndicatedCORInvalid_flg"
  [VHAL_EngTqIndicatedCORInvalid_flg] -> EngTqIndicatedCORInvalidCvt/1
  EngTqIndicatedCORCvt/1 -> halbus/36  "VHAL_EngTqIndicatedCOR_Nm"
  [VHAL_EngTqIndicatedCOR_Nm] -> EngTqIndicatedCORCvt/1
  EngTqIndicatedInvalidCvt/1 -> halbus/35  "VHAL_EngTqIndicatedInvalid_flg"
  [VHAL_EngTqIndicatedInvalid_flg] -> EngTqIndicatedInvalidCvt/1
  EngTqIndicatedCvt/1 -> halbus/34  "VHAL_EngTqIndicated_Nm"
  [VHAL_EngTqIndicated_Nm] -> EngTqIndicatedCvt/1
  EngSpdInvalidCvt/1 -> halbus/33  "VHAL_EngSpdInvalid_flg"
  [VHAL_EngSpdInvalid_flg] -> EngSpdInvalidCvt/1
  EngSpdCvt/1 -> halbus/32  "VHAL_EngSpd_erpm"
  [VHAL_EngSpd_erpm] -> EngSpdCvt/1
  EffAccelPedalPosnInvalidCvt/1 -> halbus/31  "VHAL_EffAccelPedalPosnInvalid_flg"
  [VHAL_EffAccelPedalPosnInvalid_flg] -> EffAccelPedalPosnInvalidCvt/1
  EffAccelPedalPosnCvt/1 -> halbus/30  "VHAL_EffAccelPedalPosn_pct"
  [VHAL_EffAccelPedalPosn_pct] -> EffAccelPedalPosnCvt/1
  AccelPedalPosnInvalidCvt/1 -> halbus/29  "VHAL_AccelPedalPosnInvalid_flg"
  [VHAL_AccelPedalPosnInvalid_flg] -> AccelPedalPosnInvalidCvt/1
  AccelPedalPosnCvt/1 -> halbus/28  "VHAL_AccelPedalPosn_pct"
  [VHAL_AccelPedalPosn_pct] -> AccelPedalPosnCvt/1
  LampYellowOnFltShortLowCvt/1 -> halbus/27  "VHAL_LampYellowOnFltShortLow_enum"
  [VHAL_LampYellowOnFltShortLow_enum] -> LampYellowOnFltShortLowCvt/1
  LampYellowOnFltShortHighCvt/1 -> halbus/26  "VHAL_LampYellowOnFltShortHigh_enum"
  [VHAL_LampYellowOnFltShortHigh_enum] -> LampYellowOnFltShortHighCvt/1
  LampYellowOnFltOpenCircuitCvt/1 -> halbus/25  "VHAL_LampYellowOnFltOpenCircuit_enum"
  [VHAL_LampYellowOnFltOpenCircuit_enum] -> LampYellowOnFltOpenCircuitCvt/1
  LampGreenOnFltShortLowCvt/1 -> halbus/24  "VHAL_LampGreenOnFltShortLow_enum"
  [VHAL_LampGreenOnFltShortLow_enum] -> LampGreenOnFltShortLowCvt/1
  LampGreenOnFltShortHighCvt/1 -> halbus/23  "VHAL_LampGreenOnFltShortHigh_enum"
  [VHAL_LampGreenOnFltShortHigh_enum] -> LampGreenOnFltShortHighCvt/1
  LampGreenOnFltOpenCircuitCvt/1 -> halbus/22  "VHAL_LampGreenOnFltOpenCircuit_enum"
  [VHAL_LampGreenOnFltOpenCircuit_enum] -> LampGreenOnFltOpenCircuitCvt/1
  LampBlueOnFltShortLowCvt/1 -> halbus/21  "VHAL_LampBlueOnFltShortLow_enum"
  [VHAL_LampBlueOnFltShortLow_enum] -> LampBlueOnFltShortLowCvt/1
  LampBlueOnFltShortHighCvt/1 -> halbus/20  "VHAL_LampBlueOnFltShortHigh_enum"
  [VHAL_LampBlueOnFltShortHigh_enum] -> LampBlueOnFltShortHighCvt/1
  LampBlueOnFltOpenCircuitCvt/1 -> halbus/19  "VHAL_LampBlueOnFltOpenCircuit_enum"
  [VHAL_LampBlueOnFltOpenCircuit_enum] -> LampBlueOnFltOpenCircuitCvt/1
  LampRedOnFltShortLowCvt/1 -> halbus/18  "VHAL_LampRedOnFltShortLow_enum"
  [VHAL_LampRedOnFltShortLow_enum] -> LampRedOnFltShortLowCvt/1
  LampRedOnFltShortHighCvt/1 -> halbus/17  "VHAL_LampRedOnFltShortHigh_enum"
  [VHAL_LampRedOnFltShortHigh_enum] -> LampRedOnFltShortHighCvt/1
  LampRedOnFltOpenCircuitCvt/1 -> halbus/16  "VHAL_LampRedOnFltOpenCircuit_enum"
  [VHAL_LampRedOnFltOpenCircuit_enum] -> LampRedOnFltOpenCircuitCvt/1
  OBUBuzzerOnFltShortLowCvt/1 -> halbus/15  "VHAL_OBUBuzzerOnFltShortLow_enum"
  [VHAL_OBUBuzzerOnFltShortLow_enum] -> OBUBuzzerOnFltShortLowCvt/1
  OBUBuzzerOnFltShortHighCvt/1 -> halbus/14  "VHAL_OBUBuzzerOnFltShortHigh_enum"
  [VHAL_OBUBuzzerOnFltShortHigh_enum] -> OBUBuzzerOnFltShortHighCvt/1
  OBUBuzzerOnFltOpenCircuitCvt/1 -> halbus/13  "VHAL_OBUBuzzerOnFltOpenCircuit_enum"
  [VHAL_OBUBuzzerOnFltOpenCircuit_enum] -> OBUBuzzerOnFltOpenCircuitCvt/1
  BuzzerSwOnFltShortLowCvt/1 -> halbus/12  "VHAL_BuzzerSwOnFltShortLow_enum"
  [VHAL_BuzzerSwOnFltShortLow_enum] -> BuzzerSwOnFltShortLowCvt/1
  BuzzerSwOnFltShortHighCvt/1 -> halbus/11  "VHAL_BuzzerSwOnFltShortHigh_enum"
  [VHAL_BuzzerSwOnFltShortHigh_enum] -> BuzzerSwOnFltShortHighCvt/1
  BuzzerSwOnFltOpenCircuitCvt/1 -> halbus/10  "VHAL_BuzzerSwOnFltOpenCircuit_enum"
  [VHAL_BuzzerSwOnFltOpenCircuit_enum] -> BuzzerSwOnFltOpenCircuitCvt/1
  VREF2FaultCvt/1 -> halbus/9  "VHAL_VREF2Fault_enum"
  [VHAL_VREF2Fault_enum] -> VREF2FaultCvt/1
  VREF1FaultCvt/1 -> halbus/8  "VHAL_VREF1Fault_enum"
  [VHAL_VREF1Fault_enum] -> VREF1FaultCvt/1
  ROMFaultCvt/1 -> halbus/7  "VHAL_ROMFault_enum"
  [VHAL_ROMFault_enum] -> ROMFaultCvt/1
  RAMFaultCvt/1 -> halbus/6  "VHAL_RAMFault_enum"
  [VHAL_RAMFault_enum] -> RAMFaultCvt/1
  EEPROMFaultCvt/1 -> halbus/5  "VHAL_EEPROMFault_enum"
  [VHAL_EEPROMFault_enum] -> EEPROMFaultCvt/1
  ADCFaultCvt/1 -> halbus/4  "VHAL_ADCFault_enum"
  [VHAL_ADCFault_enum] -> ADCFaultCvt/1
  AppTimeCvt/1 -> halbus/3  "VHAL_AppTime_ms"
  [VHAL_AppTime_ms] -> AppTimeCvt/1
  VbatprotVoltCvt/1 -> halbus/2  "VHAL_VbatprotVolt_V"
  [VHAL_VbatprotVolt_V] -> VbatprotVoltCvt/1
  IgnitionVoltCvt/1 -> halbus/1  "VHAL_IgnitionVolt_V"
  [VHAL_IgnitionVolt_V] -> IgnitionVoltCvt/1
  CAN2_Rx/1 -> [CAN2_Rx]
  CAN1_Rx/1 -> [CAN1_Rx]
  [CAN1_Rx] -> dHAL_IN_ECM/1(CAN1_Rx)
  [CAN1_Rx] -> dHAL_IN_ABS/1(CAN1_Rx)
  [CAN1_Rx] -> dHAL_IN_BCM/1(CAN1_Rx)
  [CAN1_Rx] -> dHAL_IN_TCM/1(CAN1_Rx)
  [CAN1_Rx] -> dHAL_IN_EPAS/1(CAN1_Rx)
  [CAN1_Rx] -> dHAL_IN_METER/1(CAN1_Rx)
  [CAN1_Rx] -> dHAL_IN_AC/1(CAN1_Rx)
  [CAN1_Rx] -> HAL_IN_EPB/1(CAN1_Rx)
  [CAN1_Rx] -> HAL_IN_VCU/1(CAN1_Rx)
  [CAN1_Rx] -> HAL_IN_HMI/1(CAN1_Rx)
  [CAN1_Rx] -> HAL_IN_CANVALID/1(CAN1_Rx)
  [CAN2_Rx] -> HAL_IN_EPM/1(CAN2_Rx)
  [CAN2_Rx] -> HAL_IN_CANVALID/2(CAN2_Rx)
  [CAN2_Rx] -> HAL_IN_RadObjDecoder/1(CAN2_Rx)
  dHAL_IN_EPAS/26(VHAL_EPSLKAStatus_enum) -> [VHAL_EPSLKAStatus_enum]
  dHAL_IN_EPAS/28(VHAL_EPSADASAbReason_enum) -> [VHAL_EPSADASAbReason_enum]
  dHAL_IN_EPAS/27(VHAL_EPSLFCStatus_enum) -> [VHAL_EPSLFCStatus_enum]
  [VHAL_EPSLFCStatus_enum] -> EPAS3RollCntCvt2/1
  EPAS3RollCntCvt2/1 -> halbus/139  "VHAL_EPSLFCStatus_enum"
  [VHAL_EPSADASAbReason_enum] -> EPAS3RollCntCvt3/1
  EPAS3RollCntCvt3/1 -> halbus/140  "VHAL_EPSADASAbReason_enum"
  [VHAL_EPSLKAStatus_enum] -> EPAS3RollCntCvt4/1
  EPAS3RollCntCvt4/1 -> halbus/138  "VHAL_EPSLKAStatus_enum"
  HAL_IN_VCU/25(VHAL_TCMGearPosnReqAllow_enum) -> [VHAL_TCMGearPosnReqAllow_enum]
  HAL_IN_VCU/26(VHAL_MSAStatus_enum) -> [VHAL_MSAStatus_enum]
  [VHAL_TCMGearPosnReqAllow_enum] -> CurDriverTqReqInvalidCvt1/1
  CurDriverTqReqInvalidCvt1/1 -> halbus/180  "VHAL_TCMGearPosnReqAllow_enum"
  [VHAL_MSAStatus_enum] -> VCU2RollCntCvt1/1
  VCU2RollCntCvt1/1 -> halbus/181  "VHAL_MSAStatus_enum"
  ViewRangeLCvt1/1 -> halbus/231  "VHAL_ViewRangeEndL_m"
  [VHAL_ViewRangeEndL_m] -> ViewRangeLCvt1/1
  ViewRangeRCvt1/1 -> halbus/233  "VHAL_ViewRangeEndR_m"
  [VHAL_ViewRangeEndR_m] -> ViewRangeRCvt1/1
  HAL_IN_EPM/16(VHAL_ViewRangeEndL_m) -> [VHAL_ViewRangeEndL_m]
  HAL_IN_EPM/18(VHAL_ViewRangeEndR_m) -> [VHAL_ViewRangeEndR_m]
  dHAL_IN_ECM/23(VHAL_OBDDriveCycAchiv_flg) -> [VHAL_OBDDriveCycAchiv_flg]
  EngRunningCvt1/1 -> halbus/50  "VHAL_OBDDriveCycAchiv_flg"
  [VHAL_OBDDriveCycAchiv_flg] -> EngRunningCvt1/1
  dHAL_IN_TCM/7(VHAL_TqConvClutchSt_enum) -> [VHAL_TqConvClutchSt_enum]
  TCMFaultStatusCvt1/1 -> halbus/107  "VHAL_TqConvClutchSt_enum"
  [VHAL_TqConvClutchSt_enum] -> TCMFaultStatusCvt1/1
  dHAL_IN_TCM/8(VHAL_TCMMILReq_flg) -> [VHAL_TCMMILReq_flg]
  TMTurbineSpdInvalidCvt1/1 -> halbus/108  "VHAL_TCMMILReq_flg"
  [VHAL_TCMMILReq_flg] -> TMTurbineSpdInvalidCvt1/1
  dHAL_IN_TCM/9(VHAL_TCMWinterMode_flg) -> [VHAL_TCMWinterMode_flg]
  TMTurbineSpdInvalidCvt2/1 -> halbus/109  "VHAL_TCMWinterMode_flg"
  [VHAL_TCMWinterMode_flg] -> TMTurbineSpdInvalidCvt2/1
  dHAL_IN_TCM/10(VHAL_TCMPowerMode_flg) -> [VHAL_TCMPowerMode_flg]
  TMTurbineSpdInvalidCvt3/1 -> halbus/110  "VHAL_TCMPowerMode_flg"
  [VHAL_TCMPowerMode_flg] -> TMTurbineSpdInvalidCvt3/1
  DriverBrakPedalOnCvt1/1 -> halbus/166  "VHAL_DriverBrakPedalOnInvalid_flg"
  [VHAL_DriverBrakPedalOnInvalid_flg] -> DriverBrakPedalOnCvt1/1
  HAL_IN_VCU/11(VHAL_DriverBrakPedalOnInvalid_flg) -> [VHAL_DriverBrakPedalOnInvalid_flg]
  HAL_IN_EPM/15(VHAL_ViewRangeStartL_m) -> [VHAL_ViewRangeStartL_m]
  HAL_IN_EPM/25(VHAL_CamNofObjects_num) -> [VHAL_CamNofObjects_num]
  TLCRCvt1/1 -> halbus/240  "VHAL_CamNofObjects_num"
  [VHAL_CamNofObjects_num] -> TLCRCvt1/1
  HAL_IN_EPM/26(VHAL_CamGoDecision_enum) -> [VHAL_CamGoDecision_enum]
  TLCRCvt2/1 -> halbus/241  "VHAL_CamGoDecision_enum"
  [VHAL_CamGoDecision_enum] -> TLCRCvt2/1
  HAL_IN_EPM/27(VHAL_CloseCarDetected_flg) -> [VHAL_CloseCarDetected_flg]
  TLCRCvt3/1 -> halbus/242  "VHAL_CloseCarDetected_flg"
  [VHAL_CloseCarDetected_flg] -> TLCRCvt3/1
  HAL_IN_EPM/28(VHAL_RightCarCutIn_flg) -> [VHAL_RightCarCutIn_flg]
  TLCRCvt4/1 -> halbus/243  "VHAL_RightCarCutIn_flg"
  [VHAL_RightCarCutIn_flg] -> TLCRCvt4/1
  HAL_IN_EPM/29(VHAL_LeftCarCutIn_flg) -> [VHAL_LeftCarCutIn_flg]
  TLCRCvt5/1 -> halbus/244  "VHAL_LeftCarCutIn_flg"
  [VHAL_LeftCarCutIn_flg] -> TLCRCvt5/1
  HAL_IN_EPM/30(VHAL_CamFSImpairedVD_flg) -> [VHAL_CamFSImpairedVD_flg]
  TLCRCvt6/1 -> halbus/245  "VHAL_CamFSImpairedVD_flg"
  [VHAL_CamFSImpairedVD_flg] -> TLCRCvt6/1
  HAL_IN_EPM/31(VHAL_CamFSLowSun_flg) -> [VHAL_CamFSLowSun_flg]
  TLCRCvt7/1 -> halbus/246  "VHAL_CamFSLowSun_flg"
  [VHAL_CamFSLowSun_flg] -> TLCRCvt7/1
  TLCRCvt8/1 -> halbus/247  "VHAL_CamFSBlurImage_flg"
  [VHAL_CamFSBlurImage_flg] -> TLCRCvt8/1
  HAL_IN_EPM/32(VHAL_CamFSBlurImage_flg) -> [VHAL_CamFSBlurImage_flg]
  HAL_IN_EPM/33(VHAL_CamFSSmearImage_flg) -> [VHAL_CamFSSmearImage_flg]
  TLCRCvt9/1 -> halbus/248  "VHAL_CamFSSmearImage_flg"
  [VHAL_CamFSSmearImage_flg] -> TLCRCvt9/1
  HAL_IN_EPM/34(VHAL_CamFSPartialBlockage_flg) -> [VHAL_CamFSPartialBlockage_flg]
  TLCRCvt10/1 -> halbus/249  "VHAL_CamFSPartialBlockage_flg"
  [VHAL_CamFSPartialBlockage_flg] -> TLCRCvt10/1
  HAL_IN_EPM/35(VHAL_CamFSFullBlockage_flg) -> [VHAL_CamFSFullBlockage_flg]
  TLCRCvt11/1 -> halbus/250  "VHAL_CamFSFullBlockage_flg"
  [VHAL_CamFSFullBlockage_flg] -> TLCRCvt11/1
  HAL_IN_EPM/36(VHAL_CamFSSplashes_flg) -> [VHAL_CamFSSplashes_flg]
  TLCRCvt12/1 -> halbus/251  "VHAL_CamFSSplashes_flg"
  [VHAL_CamFSSplashes_flg] -> TLCRCvt12/1
  HAL_IN_EPM/37(VHAL_CamFSOutofCal_flg) -> [VHAL_CamFSOutofCal_flg]
  TLCRCvt13/1 -> halbus/252  "VHAL_CamFSOutofCal_flg"
  [VHAL_CamFSOutofCal_flg] -> TLCRCvt13/1
  HAL_IN_EPM/38(VHAL_CamFSCalMisalign_flg) -> [VHAL_CamFSCalMisalign_flg]
  TLCRCvt14/1 -> halbus/253  "VHAL_CamFSCalMisalign_flg"
  [VHAL_CamFSCalMisalign_flg] -> TLCRCvt14/1
  HAL_IN_EPM/39(VHAL_CamFSSmearedspots_flg) -> [VHAL_CamFSSmearedspots_flg]
  TLCRCvt15/1 -> halbus/254  "VHAL_CamFSSmearedspots_flg"
  [VHAL_CamFSSmearedspots_flg] -> TLCRCvt15/1
  HAL_IN_EPM/40(VHAL_CamFSSpotHalosFrozen_flg) -> [VHAL_CamFSSpotHalosFrozen_flg]
  TLCRCvt16/1 -> halbus/255  "VHAL_CamFSSpotHalosFrozen_flg"
  [VHAL_CamFSSpotHalosFrozen_flg] -> TLCRCvt16/1
  HAL_IN_EPM/41(VHAL_CamFSFoggySpots_flg) -> [VHAL_CamFSFoggySpots_flg]
  TLCRCvt17/1 -> halbus/256  "VHAL_CamFSFoggySpots_flg"
  [VHAL_CamFSFoggySpots_flg] -> TLCRCvt17/1
  HAL_IN_EPM/42(VHAL_CamFSSunRay_flg) -> [VHAL_CamFSSunRay_flg]
  TLCRCvt18/1 -> halbus/257  "VHAL_CamFSSunRay_flg"
  [VHAL_CamFSSunRay_flg] -> TLCRCvt18/1
  HAL_IN_CSW/2(VHAL_HighBeamSwOn_flg) -> [VHAL_HighBeamSwOn_flg]
  HAL_IN_CSW/1(VHAL_RearFogSwOn_flg) -> [VHAL_RearFogSwOn_flg]
  [CAN1_Rx] -> HAL_IN_CSW/1(CAN1_Rx)
  ParkBrakeBindStaInvalidCvt1/1 -> halbus/154  "VHAL_RearFogSwOn_flg"
  [VHAL_RearFogSwOn_flg] -> ParkBrakeBindStaInvalidCvt1/1
  ParkBrakeBindStaInvalidCvt2/1 -> halbus/155  "VHAL_HighBeamSwOn_flg"
  [VHAL_HighBeamSwOn_flg] -> ParkBrakeBindStaInvalidCvt2/1
  HAL_IN_CANVALID/21(VHAL_CANMsgValidCSW1_flg) -> [VHAL_CANMsgValidCSW1_flg]
  CANMsgValidEPB1Cvt1/1 -> halbus/305  "VHAL_CANMsgValidCSW1_flg"
  [VHAL_CANMsgValidCSW1_flg] -> CANMsgValidEPB1Cvt1/1
  HAL_IN_CANVALID/32(VHAL_CANMsgValidEPM5_flg) -> [VHAL_CANMsgValidEPM5_flg]
  CANMsgValidEPM4Cvt1/1 -> halbus/315  "VHAL_CANMsgValidEPM4_flg"
  [VHAL_CANMsgValidEPM4_flg] -> CANMsgValidEPM4Cvt1/1
